simulink library "halin"  (R2024a)
settings: Solver=VariableStepAuto  StartTime=0.0  StopTime=10.0  RelTol=1e-3
undefined symbols (not defined in the file): KHAL_CAN3BMS1E2E_flg, KHAL_CAN3BMS6E2E_flg, TimeoutOccurred
libraries: FVT_lib x12, simulink x6, hcu_lib x1
(part 1 of 2)
settings Model: Creator=13168  LastModifiedBy=FVT22063
settings SolverCC: AlgebraicLoopSolver=TrustRegion
settings DataIOCC: SaveFormat=Array  SignalLoggingSaveFormat=ModelDataLogs  ReturnWorkspaceOutputs=off
settings OptimizationCC: BlockReduction=off  BooleanDataType=off
settings DebuggingCC: SaveWithParameterizedLinksMsg=none  UnderspecifiedInitializationDetection=Classic  MergeDetectMultiDrivingBlocksExec=none  SignalResolutionControl=TryResolveAllWithWarning  UnconnectedInputMsg=warning  UnconnectedOutputMsg=warning  UnconnectedLineMsg=warning
settings HardwareCC: TargetUnknown=on
settings ModelReferenceCC: EnableRefExpFcnMdlSchedulingChecks=on  PropagateSignalLabelsOutOfModel=off
settings RTWCC: GPUComputeCapability=3.5  DLArmComputeVersion=19.05
settings ConfigComp: CovMetricSettings=dw  CovSaveCumulativeToWorkspaceVar=on  CovSaveSingleToWorkspaceVar=on

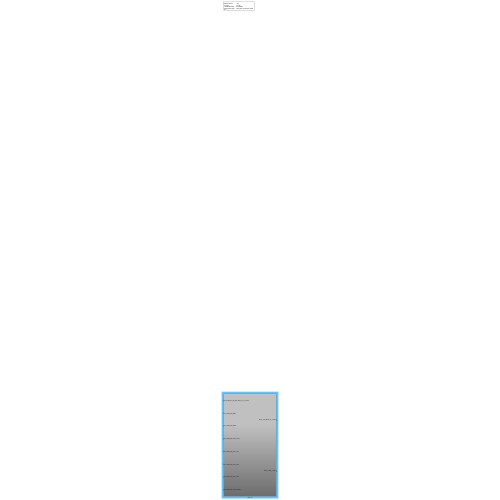
[thumbnail: Simulink's stored preview of the top-level diagram]
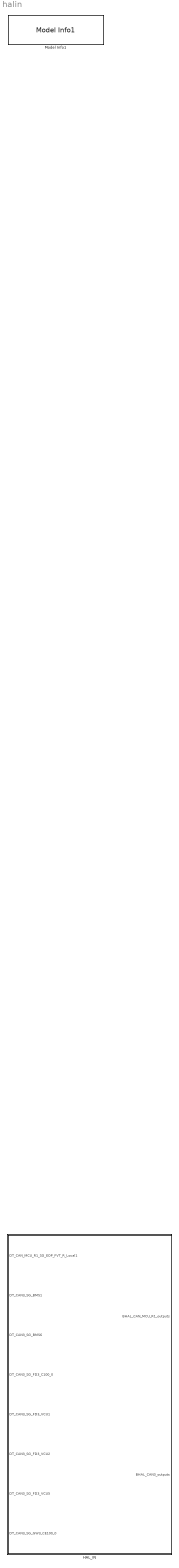
== system halin ==
  HAL_IN : Subsystem
      settings: RTWSystemCode=Nonreusable function  RTWFcnNameOpts=Use subsystem name  RTWFileNameOpts=Use subsystem name
  Model Info1 : hcu_lib/Model Info1  BlockCM=None  Frame=on  DisplayStringWithTags=|  HorizontalTextAlignment=Left  LeftAlignmentValue=0.02  SourceBlockDiagram=hcu_lib  TagMaxNumber=20
      | Model Version        : %<ModelVersion>
      | Creator                   : %<Creator>
      | Last Modified By    : %<LastModifiedBy>
      | Modification date    : %<LastModificationDate>
      settings: SourceProductName=HCU Relative Block Library

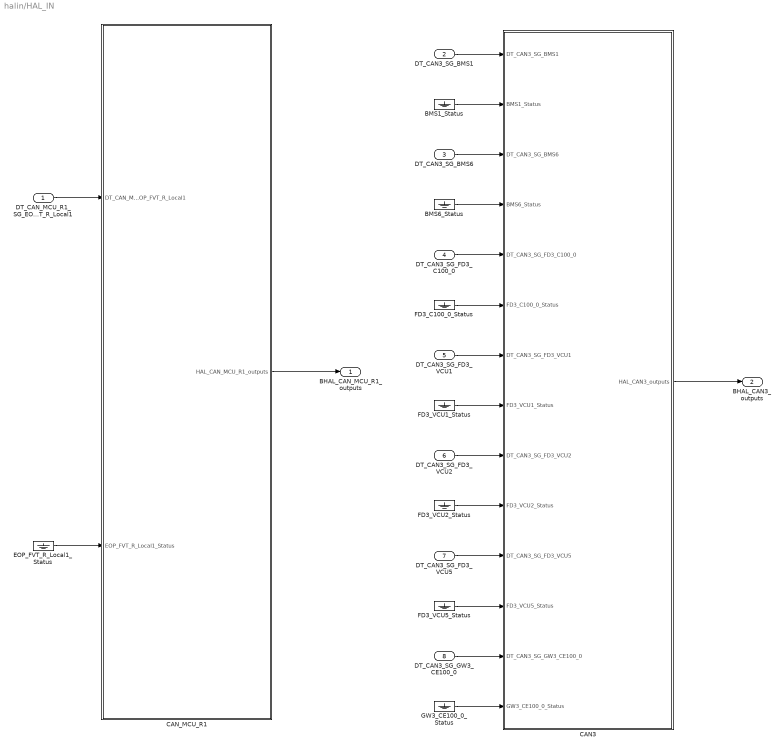
== system halin/HAL_IN ==
  DT_CAN_MCU_R1_SG_EOP_FVT_R_Local1 : Inport
  DT_CAN3_SG_BMS1 : Inport  Port=2
  DT_CAN3_SG_BMS6 : Inport  Port=3
  DT_CAN3_SG_FD3_C100_0 : Inport  Port=4
  DT_CAN3_SG_FD3_VCU1 : Inport  Port=5
  DT_CAN3_SG_FD3_VCU2 : Inport  Port=6
  DT_CAN3_SG_FD3_VCU5 : Inport  Port=7
  DT_CAN3_SG_GW3_CE100_0 : Inport  Port=8
  BMS1_Status : Ground
  BMS6_Status : Ground
  CAN3 : Subsystem
  CAN_MCU_R1 : Subsystem
  EOP_FVT_R_Local1_Status : Ground
  FD3_C100_0_Status : Ground
  FD3_VCU1_Status : Ground
  FD3_VCU2_Status : Ground
  FD3_VCU5_Status : Ground
  GW3_CE100_0_Status : Ground
  BHAL_CAN_MCU_R1_outputs : Outport  OutDataTypeStr=Bus: BHAL_CAN_MCU_R1_outputs
  BHAL_CAN3_outputs : Outport  Port=2  OutDataTypeStr=Bus: BHAL_CAN3_outputs
  wires:
  GW3_CE100_0_Status/1 -> CAN3/14(GW3_CE100_0_Status)
  DT_CAN3_SG_GW3_CE100_0/1 -> CAN3/13(DT_CAN3_SG_GW3_CE100_0)
  FD3_VCU5_Status/1 -> CAN3/12(FD3_VCU5_Status)
  DT_CAN3_SG_FD3_VCU5/1 -> CAN3/11(DT_CAN3_SG_FD3_VCU5)
  DT_CAN3_SG_FD3_VCU2/1 -> CAN3/9(DT_CAN3_SG_FD3_VCU2)
  FD3_VCU2_Status/1 -> CAN3/10(FD3_VCU2_Status)
  FD3_VCU1_Status/1 -> CAN3/8(FD3_VCU1_Status)
  FD3_C100_0_Status/1 -> CAN3/6(FD3_C100_0_Status)
  DT_CAN3_SG_FD3_VCU1/1 -> CAN3/7(DT_CAN3_SG_FD3_VCU1)
  DT_CAN3_SG_FD3_C100_0/1 -> CAN3/5(DT_CAN3_SG_FD3_C100_0)
  DT_CAN3_SG_BMS6/1 -> CAN3/3(DT_CAN3_SG_BMS6)
  BMS6_Status/1 -> CAN3/4(BMS6_Status)
  CAN3/1(HAL_CAN3_outputs) -> BHAL_CAN3_outputs/1
  BMS1_Status/1 -> CAN3/2(BMS1_Status)
  CAN_MCU_R1/1(HAL_CAN_MCU_R1_outputs) -> BHAL_CAN_MCU_R1_outputs/1
  EOP_FVT_R_Local1_Status/1 -> CAN_MCU_R1/2(EOP_FVT_R_Local1_Status)
  DT_CAN3_SG_BMS1/1 -> CAN3/1(DT_CAN3_SG_BMS1)
  DT_CAN_MCU_R1_SG_EOP_FVT_R_Local1/1 -> CAN_MCU_R1/1(DT_CAN_MCU_R1_SG_EOP_FVT_R_Local1)

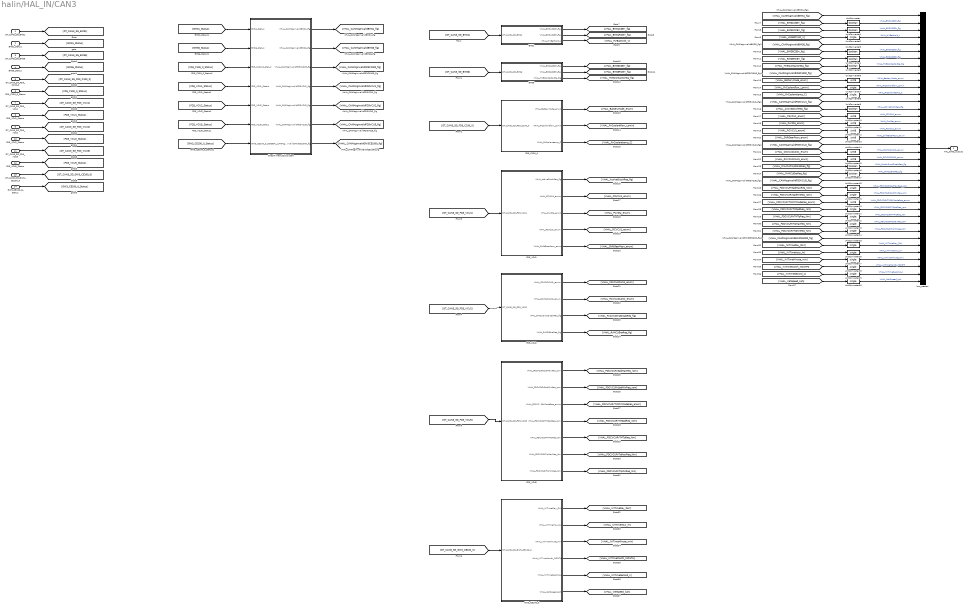
== system halin/HAL_IN/CAN3 ==
  DT_CAN3_SG_BMS1 : Inport
  BMS1_Status : Inport  Port=2
  DT_CAN3_SG_BMS6 : Inport  Port=3
  BMS6_Status : Inport  Port=4
  DT_CAN3_SG_FD3_C100_0 : Inport  Port=5
  FD3_C100_0_Status : Inport  Port=6
  DT_CAN3_SG_FD3_VCU1 : Inport  Port=7
  FD3_VCU1_Status : Inport  Port=8
  DT_CAN3_SG_FD3_VCU2 : Inport  Port=9
  FD3_VCU2_Status : Inport  Port=10
  DT_CAN3_SG_FD3_VCU5 : Inport  Port=11
  FD3_VCU5_Status : Inport  Port=12
  DT_CAN3_SG_GW3_CE100_0 : Inport  Port=13
  GW3_CE100_0_Status : Inport  Port=14
  BMS1 : Subsystem
  BMS6 : Subsystem
  CheckTimeoutSubsystem : Subsystem
  FD3_C100_0 : Subsystem
  FD3_VCU1 : Subsystem
  FD3_VCU2 : Subsystem
  FD3_VCU5 : Subsystem
  GW3_CE100_0 : Subsystem
  UnitConverter{,1,3..5,9,16..17} (8 alike) : DataTypeConversion  OutDataTypeStr=boolean  SaturateOnIntegerOverflow=off  RndMeth=Floor
  UnitConverter{6,10..15,20} (8 alike) : DataTypeConversion  OutDataTypeStr=uint8  SaturateOnIntegerOverflow=off  RndMeth=Floor
  UnitConverter{2,7..8,18..19,21..30} (15 alike) : DataTypeConversion  OutDataTypeStr=single  SaturateOnIntegerOverflow=off  RndMeth=Floor
  bus_creator : BusCreator  Inputs=38  OutDataTypeStr=Bus: BHAL_CAN3_outputs  NonVirtualBus=on
  HAL_CAN3_outputs : Outport
  wires:
  BMS1_Status/1 -> [BMS1_Status]
  DT_CAN3_SG_BMS1/1 -> [DT_CAN3_SG_BMS1]
  BMS6_Status/1 -> [BMS6_Status]
  DT_CAN3_SG_BMS6/1 -> [DT_CAN3_SG_BMS6]
  FD3_C100_0_Status/1 -> [FD3_C100_0_Status]
  DT_CAN3_SG_FD3_C100_0/1 -> [DT_CAN3_SG_FD3_C100_0]
  FD3_VCU1_Status/1 -> [FD3_VCU1_Status]
  DT_CAN3_SG_FD3_VCU1/1 -> [DT_CAN3_SG_FD3_VCU1]
  FD3_VCU2_Status/1 -> [FD3_VCU2_Status]
  DT_CAN3_SG_FD3_VCU2/1 -> [DT_CAN3_SG_FD3_VCU2]
  FD3_VCU5_Status/1 -> [FD3_VCU5_Status]
  DT_CAN3_SG_FD3_VCU5/1 -> [DT_CAN3_SG_FD3_VCU5]
  GW3_CE100_0_Status/1 -> [GW3_CE100_0_Status]
  DT_CAN3_SG_GW3_CE100_0/1 -> [DT_CAN3_SG_GW3_CE100_0]
  [BMS1_Status] -> CheckTimeoutSubsystem/1(BMS1_Status)
  [BMS6_Status] -> CheckTimeoutSubsystem/2(BMS6_Status)
  [FD3_C100_0_Status] -> CheckTimeoutSubsystem/3(FD3_C100_0_Status)
  [FD3_VCU1_Status] -> CheckTimeoutSubsystem/4(FD3_VCU1_Status)
  [FD3_VCU2_Status] -> CheckTimeoutSubsystem/5(FD3_VCU2_Status)
  [FD3_VCU5_Status] -> CheckTimeoutSubsystem/6(FD3_VCU5_Status)
  [GW3_CE100_0_Status] -> CheckTimeoutSubsystem/7(GW3_CE100_0_Status)
  CheckTimeoutSubsystem/1(VHAL_CANMsgInvalidBMS1_flg) -> [VHAL_CANMsgInvalidBMS1_flg]
  CheckTimeoutSubsystem/2(VHAL_CANMsgInvalidBMS6_flg) -> [VHAL_CANMsgInvalidBMS6_flg]
  CheckTimeoutSubsystem/3(VHAL_CANMsgInvalidFD3C1000_flg) -> [VHAL_CANMsgInvalidFD3C1000_flg]
  CheckTimeoutSubsystem/4(VHAL_CANMsgInvalidFD3VCU1_flg) -> [VHAL_CANMsgInvalidFD3VCU1_flg]
  CheckTimeoutSubsystem/5(VHAL_CANMsgInvalidFD3VCU2_flg) -> [VHAL_CANMsgInvalidFD3VCU2_flg]
  CheckTimeoutSubsystem/6(VHAL_CANMsgInvalidFD3VCU5_flg) -> [VHAL_CANMsgInvalidFD3VCU5_flg]
  CheckTimeoutSubsystem/7(VHAL_CANMsgInvalidGW3CE1000_flg) -> [VHAL_CANMsgInvalidGW3CE1000_flg]
  [DT_CAN3_SG_BMS1] -> BMS1/1(DT_CAN3_SG_BMS1)
  [DT_CAN3_SG_BMS6] -> BMS6/1(DT_CAN3_SG_BMS6)
  [DT_CAN3_SG_FD3_C100_0] -> FD3_C100_0/1(DT_CAN3_SG_FD3_C100_0)
  [DT_CAN3_SG_FD3_VCU1] -> FD3_VCU1/1(DT_CAN3_SG_FD3_VCU1)
  [DT_CAN3_SG_FD3_VCU2] -> FD3_VCU2/1(DT_CAN3_SG_FD3_VCU2)
  [DT_CAN3_SG_FD3_VCU5] -> FD3_VCU5/1(DT_CAN3_SG_FD3_VCU5)
  [DT_CAN3_SG_GW3_CE100_0] -> GW3_CE100_0/1(DT_CAN3_SG_GW3_CE100_0)
  bus_creator/1 -> HAL_CAN3_outputs/1
  [VHAL_CANMsgInvalidBMS1_flg] -> bus_creator/1
  BMS1/1(VHAL_BMS1CSErr_flg) -> [VHAL_BMS1CSErr_flg]
  UnitConverter/1 -> bus_creator/2  "VHAL_BMS1CSErr_flg"
  [VHAL_BMS1CSErr_flg] -> UnitConverter/1
  BMS1/2(VHAL_BMS1RCErr_flg) -> [VHAL_BMS1RCErr_flg]
  UnitConverter1/1 -> bus_creator/3  "VHAL_BMS1RCErr_flg"
  [VHAL_BMS1RCErr_flg] -> UnitConverter1/1
  BMS1/3(VHAL_HVBattVolt_V) -> [VHAL_HVBattVolt_V]
  UnitConverter2/1 -> bus_creator/4  "VHAL_HVBattVolt_V"
  [VHAL_HVBattVolt_V] -> UnitConverter2/1
  [VHAL_CANMsgInvalidBMS6_flg] -> bus_creator/5
  BMS6/1(VHAL_BMS6CSErr_flg) -> [VHAL_BMS6CSErr_flg]
  UnitConverter3/1 -> bus_creator/6  "VHAL_BMS6CSErr_flg"
  [VHAL_BMS6CSErr_flg] -> UnitConverter3/1
  BMS6/2(VHAL_BMS6RCErr_flg) -> [VHAL_BMS6RCErr_flg]
  UnitConverter4/1 -> bus_creator/7  "VHAL_BMS6RCErr_flg"
  [VHAL_BMS6RCErr_flg] -> UnitConverter4/1
  BMS6/3(VHAL_HVBContactorSta_flg) -> [VHAL_HVBContactorSta_flg]
  UnitConverter5/1 -> bus_creator/8  "VHAL_HVBContactorSta_flg"
  [VHAL_HVBContactorSta_flg] -> UnitConverter5/1
  [VHAL_CANMsgInvalidFD3C1000_flg] -> bus_creator/9
  FD3_C100_0/1(VHAL_BatteryMode_enum) -> [VHAL_BatteryMode_enum]
  UnitConverter6/1 -> bus_creator/10  "VHAL_BatteryMode_enum"
  [VHAL_BatteryMode_enum] -> UnitConverter6/1
  FD3_C100_0/2(VHAL_RrCoolantflow_Lpmin) -> [VHAL_RrCoolantflow_Lpmin]
  UnitConverter7/1 -> bus_creator/11  "VHAL_RrCoolantflow_Lpmin"
  [VHAL_RrCoolantflow_Lpmin] -> UnitConverter7/1
  FD3_C100_0/3(VHAL_RrCoolanttemp_C) -> [VHAL_RrCoolanttemp_C]
  UnitConverter8/1 -> bus_creator/12  "VHAL_RrCoolanttemp_C"
  [VHAL_RrCoolanttemp_C] -> UnitConverter8/1
  [VHAL_CANMsgInvalidFD3VCU1_flg] -> bus_creator/13
  FD3_VCU1/1(VHAL_ActiveDischReq_flg) -> [VHAL_ActiveDischReq_flg]
  UnitConverter9/1 -> bus_creator/14  "VHAL_ActiveDischReq_flg"
  [VHAL_ActiveDischReq_flg] -> UnitConverter9/1
  FD3_VCU1/2(VHAL_CSVCU1_enum) -> [VHAL_CSVCU1_enum]
  UnitConverter10/1 -> bus_creator/15  "VHAL_CSVCU1_enum"
  [VHAL_CSVCU1_enum] -> UnitConverter10/1
  FD3_VCU1/3(VHAL_PwrSta_enum) -> [VHAL_PwrSta_enum]
  UnitConverter11/1 -> bus_creator/16  "VHAL_PwrSta_enum"
  [VHAL_PwrSta_enum] -> UnitConverter11/1
  FD3_VCU1/4(VHAL_RCVCU1_enum) -> [VHAL_RCVCU1_enum]
  UnitConverter12/1 -> bus_creator/17  "VHAL_RCVCU1_enum"
  [VHAL_RCVCU1_enum] -> UnitConverter12/1
  FD3_VCU1/5(VHAL_ShiftGearPosn_enum) -> [VHAL_ShiftGearPosn_enum]
  UnitConverter13/1 -> bus_creator/18  "VHAL_ShiftGearPosn_enum"
  [VHAL_ShiftGearPosn_enum] -> UnitConverter13/1
  [VHAL_CANMsgInvalidFD3VCU2_flg] -> bus_creator/19
  FD3_VCU2/1(VHAL_CSVCU2CAN1_enum) -> [VHAL_CSVCU2CAN1_enum]
  UnitConverter14/1 -> bus_creator/20  "VHAL_CSVCU2CAN1_enum"
  [VHAL_CSVCU2CAN1_enum] -> UnitConverter14/1
  FD3_VCU2/2(VHAL_RCVCU2CAN1_enum) -> [VHAL_RCVCU2CAN1_enum]
  UnitConverter15/1 -> bus_creator/21  "VHAL_RCVCU2CAN1_enum"
  [VHAL_RCVCU2CAN1_enum] -> UnitConverter15/1
  FD3_VCU2/3(VHAL_RrActvDmpDisabReq_flg) -> [VHAL_RrActvDmpDisabReq_flg]
  UnitConverter16/1 -> bus_creator/22  "VHAL_RrActvDmpDisabReq_flg"
  [VHAL_RrActvDmpDisabReq_flg] -> UnitConverter16/1
  FD3_VCU2/4(VHAL_RrMCUEnaReq_flg) -> [VHAL_RrMCUEnaReq_flg]
  UnitConverter17/1 -> bus_creator/23  "VHAL_RrMCUEnaReq_flg"
  [VHAL_RrMCUEnaReq_flg] -> UnitConverter17/1
  [VHAL_CANMsgInvalidFD3VCU5_flg] -> bus_creator/24
  FD3_VCU5/1(VHAL_FDCVCURrSpdMaxReq_rpm) -> [VHAL_FDCVCURrSpdMaxReq_rpm]
  UnitConverter18/1 -> bus_creator/25  "VHAL_FDCVCURrSpdMaxReq_rpm"
  [VHAL_FDCVCURrSpdMaxReq_rpm] -> UnitConverter18/1
  FD3_VCU5/2(VHAL_FDCVCURrSpdMinReq_rpm) -> [VHAL_FDCVCURrSpdMinReq_rpm]
  UnitConverter19/1 -> bus_creator/26  "VHAL_FDCVCURrSpdMinReq_rpm"
  [VHAL_FDCVCURrSpdMinReq_rpm] -> UnitConverter19/1
  FD3_VCU5/3(VHAL_FDCVCURrTMCtrlModeReq_enum) -> [VHAL_FDCVCURrTMCtrlModeReq_enum]
  UnitConverter20/1 -> bus_creator/27  "VHAL_FDCVCURrTMCtrlModeReq_enum"
  [VHAL_FDCVCURrTMCtrlModeReq_enum] -> UnitConverter20/1
  FD3_VCU5/4(VHAL_FDCVCURrTMSpdReq_rpm) -> [VHAL_FDCVCURrTMSpdReq_rpm]
  UnitConverter21/1 -> bus_creator/28  "VHAL_FDCVCURrTMSpdReq_rpm"
  [VHAL_FDCVCURrTMSpdReq_rpm] -> UnitConverter21/1
  FD3_VCU5/5(VHAL_FDCVCURrTMTqReq_Nm) -> [VHAL_FDCVCURrTMTqReq_Nm]
  UnitConverter22/1 -> bus_creator/29  "VHAL_FDCVCURrTMTqReq_Nm"
  [VHAL_FDCVCURrTMTqReq_Nm] -> UnitConverter22/1
  FD3_VCU5/6(VHAL_FDCVCURrTqMaxReq_Nm) -> [VHAL_FDCVCURrTqMaxReq_Nm]
  UnitConverter23/1 -> bus_creator/30  "VHAL_FDCVCURrTqMaxReq_Nm"
  [VHAL_FDCVCURrTqMaxReq_Nm] -> UnitConverter23/1
  FD3_VCU5/7(VHAL_FDCVCURrTqMinReq_Nm) -> [VHAL_FDCVCURrTqMinReq_Nm]
  UnitConverter24/1 -> bus_creator/31  "VHAL_FDCVCURrTqMinReq_Nm"
  [VHAL_FDCVCURrTqMinReq_Nm] -> UnitConverter24/1
  [VHAL_CANMsgInvalidGW3CE1000_flg] -> bus_creator/32
  GW3_CE100_0/1(VHAL_IVITimeDay_DAY) -> [VHAL_IVITimeDay_DAY]
  UnitConverter25/1 -> bus_creator/33  "VHAL_IVITimeDay_DAY"
  [VHAL_IVITimeDay_DAY] -> UnitConverter25/1
  GW3_CE100_0/2(VHAL_IVITimeHour_hr) -> [VHAL_IVITimeHour_hr]
  UnitConverter26/1 -> bus_creator/34  "VHAL_IVITimeHour_hr"
  [VHAL_IVITimeHour_hr] -> UnitConverter26/1
  GW3_CE100_0/3(VHAL_IVITimeMinute_min) -> [VHAL_IVITimeMinute_min]
  UnitConverter27/1 -> bus_creator/35  "VHAL_IVITimeMinute_min"
  [VHAL_IVITimeMinute_min] -> UnitConverter27/1
  GW3_CE100_0/4(VHAL_IVITimeMonth_MONTH) -> [VHAL_IVITimeMonth_MONTH]
  UnitConverter28/1 -> bus_creator/36  "VHAL_IVITimeMonth_MONTH"
  [VHAL_IVITimeMonth_MONTH] -> UnitConverter28/1
  GW3_CE100_0/5(VHAL_IVITimeSecond_s) -> [VHAL_IVITimeSecond_s]
  UnitConverter29/1 -> bus_creator/37  "VHAL_IVITimeSecond_s"
  [VHAL_IVITimeSecond_s] -> UnitConverter29/1
  GW3_CE100_0/6(VHAL_VehSpeed_kph) -> [VHAL_VehSpeed_kph]
  UnitConverter30/1 -> bus_creator/38  "VHAL_VehSpeed_kph"
  [VHAL_VehSpeed_kph] -> UnitConverter30/1

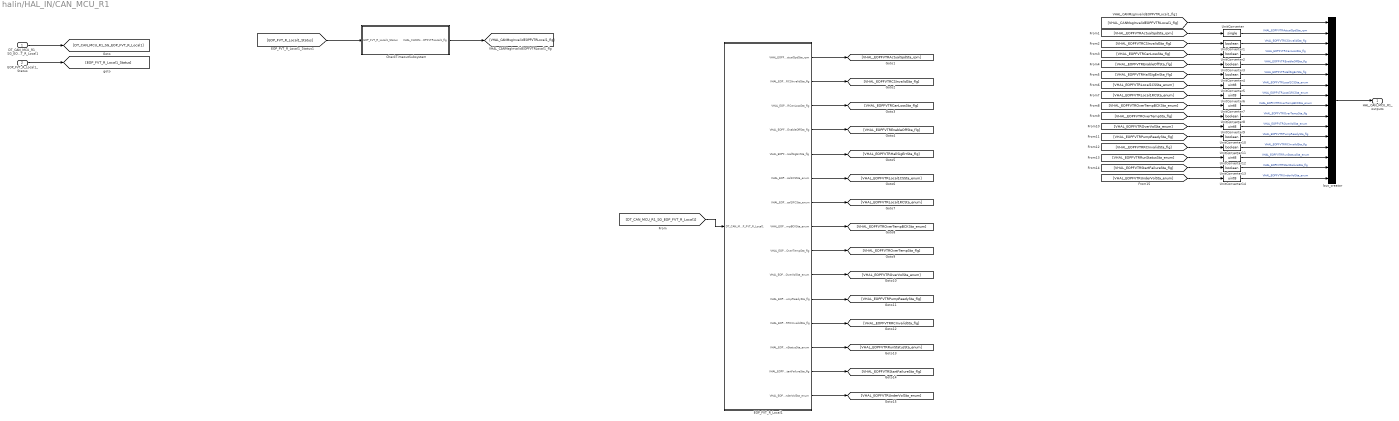
== system halin/HAL_IN/CAN_MCU_R1 ==
  DT_CAN_MCU_R1_SG_EOP_FVT_R_Local1 : Inport
  EOP_FVT_R_Local1_Status : Inport  Port=2
  CheckTimeoutSubsystem : Subsystem
  EOP_FVT_R_Local1 : Subsystem
  UnitConverter : DataTypeConversion  OutDataTypeStr=single  SaturateOnIntegerOverflow=off  RndMeth=Floor
  UnitConverter{1..4,8,10..11,13} (8 alike) : DataTypeConversion  OutDataTypeStr=boolean  SaturateOnIntegerOverflow=off  RndMeth=Floor
  UnitConverter{5..7,9,12,14} (6 alike) : DataTypeConversion  OutDataTypeStr=uint8  SaturateOnIntegerOverflow=off  RndMeth=Floor
  bus_creator : BusCreator  Inputs=16  OutDataTypeStr=Bus: BHAL_CAN_MCU_R1_outputs  NonVirtualBus=on
  HAL_CAN_MCU_R1_outputs : Outport
  wires:
  EOP_FVT_R_Local1_Status/1 -> [EOP_FVT_R_Local1_Status]
  DT_CAN_MCU_R1_SG_EOP_FVT_R_Local1/1 -> [DT_CAN_MCU_R1_SG_EOP_FVT_R_Local1]
  [EOP_FVT_R_Local1_Status] -> CheckTimeoutSubsystem/1(EOP_FVT_R_Local1_Status)
  CheckTimeoutSubsystem/1(VHAL_CANMsgInvalidEOPFVTRLocal1_flg) -> [VHAL_CANMsgInvalidEOPFVTRLocal1_flg]
  [DT_CAN_MCU_R1_SG_EOP_FVT_R_Local1] -> EOP_FVT_R_Local1/1(DT_CAN_MCU_R1_SG_EOP_FVT_R_Local1)
  bus_creator/1 -> HAL_CAN_MCU_R1_outputs/1
  [VHAL_CANMsgInvalidEOPFVTRLocal1_flg] -> bus_creator/1
  EOP_FVT_R_Local1/1(VHAL_EOPFVTRActualSpdSta_rpm) -> [VHAL_EOPFVTRActualSpdSta_rpm]
  UnitConverter/1 -> bus_creator/2  "VHAL_EOPFVTRActualSpdSta_rpm"
  [VHAL_EOPFVTRActualSpdSta_rpm] -> UnitConverter/1
  EOP_FVT_R_Local1/2(VHAL_EOPFVTRCSInvalidSta_flg) -> [VHAL_EOPFVTRCSInvalidSta_flg]
  UnitConverter1/1 -> bus_creator/3  "VHAL_EOPFVTRCSInvalidSta_flg"
  [VHAL_EOPFVTRCSInvalidSta_flg] -> UnitConverter1/1
  EOP_FVT_R_Local1/3(VHAL_EOPFVTRCanLossSta_flg) -> [VHAL_EOPFVTRCanLossSta_flg]
  UnitConverter2/1 -> bus_creator/4  "VHAL_EOPFVTRCanLossSta_flg"
  [VHAL_EOPFVTRCanLossSta_flg] -> UnitConverter2/1
  EOP_FVT_R_Local1/4(VHAL_EOPFVTREnableOffSta_flg) -> [VHAL_EOPFVTREnableOffSta_flg]
  UnitConverter3/1 -> bus_creator/5  "VHAL_EOPFVTREnableOffSta_flg"
  [VHAL_EOPFVTREnableOffSta_flg] -> UnitConverter3/1
  EOP_FVT_R_Local1/5(VHAL_EOPFVTRHallSigErrSta_flg) -> [VHAL_EOPFVTRHallSigErrSta_flg]
  UnitConverter4/1 -> bus_creator/6  "VHAL_EOPFVTRHallSigErrSta_flg"
  [VHAL_EOPFVTRHallSigErrSta_flg] -> UnitConverter4/1
  EOP_FVT_R_Local1/6(VHAL_EOPFVTRLocal1CSSta_enum) -> [VHAL_EOPFVTRLocal1CSSta_enum]
  UnitConverter5/1 -> bus_creator/7  "VHAL_EOPFVTRLocal1CSSta_enum"
  [VHAL_EOPFVTRLocal1CSSta_enum] -> UnitConverter5/1
  EOP_FVT_R_Local1/7(VHAL_EOPFVTRLocal1RCSta_enum) -> [VHAL_EOPFVTRLocal1RCSta_enum]
  UnitConverter6/1 -> bus_creator/8  "VHAL_EOPFVTRLocal1RCSta_enum"
  [VHAL_EOPFVTRLocal1RCSta_enum] -> UnitConverter6/1
  EOP_FVT_R_Local1/8(VHAL_EOPFVTROverTempBCKSta_enum) -> [VHAL_EOPFVTROverTempBCKSta_enum]
  UnitConverter7/1 -> bus_creator/9  "VHAL_EOPFVTROverTempBCKSta_enum"
  [VHAL_EOPFVTROverTempBCKSta_enum] -> UnitConverter7/1
  EOP_FVT_R_Local1/9(VHAL_EOPFVTROverTempSta_flg) -> [VHAL_EOPFVTROverTempSta_flg]
  UnitConverter8/1 -> bus_creator/10  "VHAL_EOPFVTROverTempSta_flg"
  [VHAL_EOPFVTROverTempSta_flg] -> UnitConverter8/1
  EOP_FVT_R_Local1/10(VHAL_EOPFVTROverVolSta_enum) -> [VHAL_EOPFVTROverVolSta_enum]
  UnitConverter9/1 -> bus_creator/11  "VHAL_EOPFVTROverVolSta_enum"
  [VHAL_EOPFVTROverVolSta_enum] -> UnitConverter9/1
  EOP_FVT_R_Local1/11(VHAL_EOPFVTRPumpReadySta_flg) -> [VHAL_EOPFVTRPumpReadySta_flg]
  UnitConverter10/1 -> bus_creator/12  "VHAL_EOPFVTRPumpReadySta_flg"
  [VHAL_EOPFVTRPumpReadySta_flg] -> UnitConverter10/1
  EOP_FVT_R_Local1/12(VHAL_EOPFVTRRCInvalidSta_flg) -> [VHAL_EOPFVTRRCInvalidSta_flg]
  UnitConverter11/1 -> bus_creator/13  "VHAL_EOPFVTRRCInvalidSta_flg"
  [VHAL_EOPFVTRRCInvalidSta_flg] -> UnitConverter11/1
  EOP_FVT_R_Local1/13(VHAL_EOPFVTRRunStatusSta_enum) -> [VHAL_EOPFVTRRunStatusSta_enum]
  UnitConverter12/1 -> bus_creator/14  "VHAL_EOPFVTRRunStatusSta_enum"
  [VHAL_EOPFVTRRunStatusSta_enum] -> UnitConverter12/1
  EOP_FVT_R_Local1/14(VHAL_EOPFVTRStartFailureSta_flg) -> [VHAL_EOPFVTRStartFailureSta_flg]
  UnitConverter13/1 -> bus_creator/15  "VHAL_EOPFVTRStartFailureSta_flg"
  [VHAL_EOPFVTRStartFailureSta_flg] -> UnitConverter13/1
  EOP_FVT_R_Local1/15(VHAL_EOPFVTRUnderVolSta_enum) -> [VHAL_EOPFVTRUnderVolSta_enum]
  UnitConverter14/1 -> bus_creator/16  "VHAL_EOPFVTRUnderVolSta_enum"
  [VHAL_EOPFVTRUnderVolSta_enum] -> UnitConverter14/1

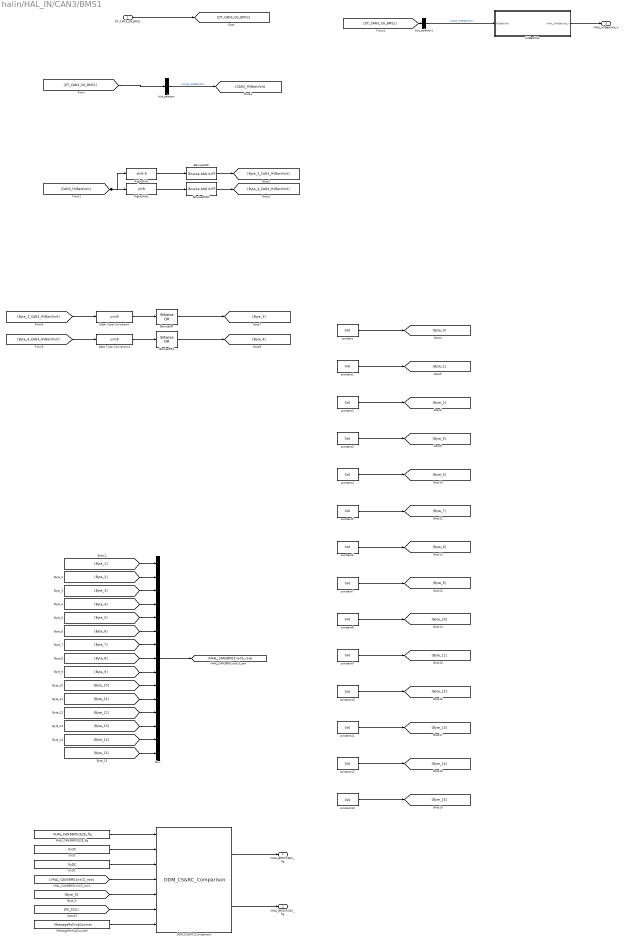
== system halin/HAL_IN/CAN3/BMS1 ==
  DT_CAN3_SG_BMS1 : Inport
  0x3C : Constant  Value=0x3C
  0xDC : Constant  Value=0xDC
  BitwiseAND : simulink/Logic and Bit Operations/Bitwise Operator  logicop=AND  UseBitMask=on  BitMask=0xFF  BitMaskRealWorld=Stored Integer
  BitwiseAND1 : simulink/Logic and Bit Operations/Bitwise Operator  logicop=AND  UseBitMask=on  BitMask=0xFF  BitMaskRealWorld=Stored Integer
  BitwiseOR : simulink/Logic and Bit Operations/Bitwise Operator  logicop=OR  UseBitMask=off  BitMask=bin2dec('11011001')  BitMaskRealWorld=Stored Integer
  BitwiseOR1 : simulink/Logic and Bit Operations/Bitwise Operator  logicop=OR  UseBitMask=off  BitMask=bin2dec('11011001')  BitMaskRealWorld=Stored Integer
  DDM_CS&RC_Comparison : FVT_lib/hal/DDM_CS&RC_Comparison  MsgCycleTime=10
  Data Type Conversion : DataTypeConversion  OutDataTypeStr=uint8  SaturateOnIntegerOverflow=off  RndMeth=Floor
  Data Type Conversion1 : DataTypeConversion  OutDataTypeStr=uint8  SaturateOnIntegerOverflow=off  RndMeth=Floor
  HVBattVolt : Subsystem
  KHAL_CAN3BMS1E2E_flg : Constant  Value=KHAL_CAN3BMS1E2E_flg
  MessageRollingCounter : FVT_lib/hal/MessageRollingCounter  CounterMAX=14  task_time_ms=5  msg_time_ms=10
  Mux : Mux  Inputs=15
  RightShift : ArithShift  BitShiftNumber=8
  RightShift1 : ArithShift
  bus_selector : BusSelector  OutputSignals=CAN3_HVBattVolt
  bus_selector1 : BusSelector  OutputSignals=CAN3_HVBattVolt
  constant{,1..13} (14 alike) : Constant  Value=0x0  OutDataTypeStr=uint8
  VHAL_BMS1CSErr_flg : Outport
  VHAL_BMS1RCErr_flg : Outport  Port=2
  VHAL_HVBattVolt_V : Outport  Port=3
  wires:
  DT_CAN3_SG_BMS1/1 -> [DT_CAN3_SG_BMS1]
  [DT_CAN3_SG_BMS1] -> bus_selector/1
  bus_selector/1 -> [CAN3_HVBattVolt]  "<CAN3_HVBattVolt>"
  [CAN3_HVBattVolt] -> RightShift/1, RightShift1/1
  RightShift/1 -> BitwiseAND/1
  BitwiseAND/1 -> [Byte_3_CAN3_HVBattVolt]
  RightShift1/1 -> BitwiseAND1/1
  BitwiseAND1/1 -> [Byte_4_CAN3_HVBattVolt]
  constant/1 -> [Byte_0]
  constant1/1 -> [Byte_1]
  constant2/1 -> [Byte_2]
  Data Type Conversion/1 -> BitwiseOR/1
  [Byte_3_CAN3_HVBattVolt] -> Data Type Conversion/1
  BitwiseOR/1 -> [Byte_3]
  Data Type Conversion1/1 -> BitwiseOR1/1
  [Byte_4_CAN3_HVBattVolt] -> Data Type Conversion1/1
  BitwiseOR1/1 -> [Byte_4]
  constant3/1 -> [Byte_5]
  constant4/1 -> [Byte_6]
  constant5/1 -> [Byte_7]
  constant6/1 -> [Byte_8]
  constant7/1 -> [Byte_9]
  constant8/1 -> [Byte_10]
  constant9/1 -> [Byte_11]
  constant10/1 -> [Byte_12]
  constant11/1 -> [Byte_13]
  constant12/1 -> [Byte_14]
  constant13/1 -> [Byte_15]
  [Byte_1] -> Mux/1
  [Byte_2] -> Mux/2
  [Byte_3] -> Mux/3
  [Byte_4] -> Mux/4
  [Byte_5] -> Mux/5
  [Byte_6] -> Mux/6
  [Byte_7] -> Mux/7
  [Byte_8] -> Mux/8
  [Byte_9] -> Mux/9
  [Byte_10] -> Mux/10
  [Byte_11] -> Mux/11
  [Byte_12] -> Mux/12
  [Byte_13] -> Mux/13
  [Byte_14] -> Mux/14
  [Byte_15] -> Mux/15
  Mux/1 -> [VHAL_CAN3BMS1noCS_raw]
  KHAL_CAN3BMS1E2E_flg/1 -> DDM_CS&RC_Comparison/1
  0x3C/1 -> DDM_CS&RC_Comparison/2
  0xDC/1 -> DDM_CS&RC_Comparison/3
  [VHAL_CAN3BMS1noCS_raw] -> DDM_CS&RC_Comparison/4
  [Byte_0] -> DDM_CS&RC_Comparison/5
  [RC_ECU] -> DDM_CS&RC_Comparison/6
  MessageRollingCounter/1 -> DDM_CS&RC_Comparison/7
  DDM_CS&RC_Comparison/1 -> VHAL_BMS1CSErr_flg/1
  DDM_CS&RC_Comparison/2 -> VHAL_BMS1RCErr_flg/1
  [DT_CAN3_SG_BMS1] -> bus_selector1/1
  bus_selector1/1 -> HVBattVolt/1(HVBattVolt)  "<CAN3_HVBattVolt>"
  HVBattVolt/1(VHAL_HVBattVolt_V) -> VHAL_HVBattVolt_V/1

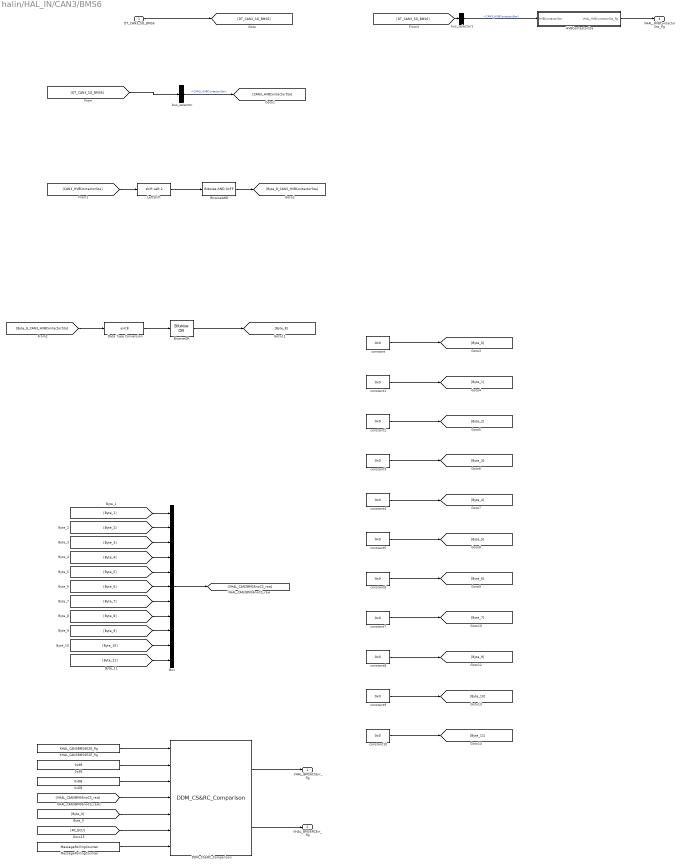
== system halin/HAL_IN/CAN3/BMS6 ==
  DT_CAN3_SG_BMS6 : Inport
  0x3B : Constant  Value=0x3B
  0xDB : Constant  Value=0xDB
  BitwiseAND : simulink/Logic and Bit Operations/Bitwise Operator  logicop=AND  UseBitMask=on  BitMask=0xFF  BitMaskRealWorld=Stored Integer
  BitwiseOR : simulink/Logic and Bit Operations/Bitwise Operator  logicop=OR  UseBitMask=off  BitMask=bin2dec('11011001')  BitMaskRealWorld=Stored Integer
  DDM_CS&RC_Comparison : FVT_lib/hal/DDM_CS&RC_Comparison  MsgCycleTime=100
  Data Type Conversion : DataTypeConversion  OutDataTypeStr=uint8  SaturateOnIntegerOverflow=off  RndMeth=Floor
  HVBContactorSta : Subsystem
  KHAL_CAN3BMS6E2E_flg : Constant  Value=KHAL_CAN3BMS6E2E_flg
  LeftShift : ArithShift  BitShiftNumber=2  BitShiftDirection=Left
  MessageRollingCounter : FVT_lib/hal/MessageRollingCounter  CounterMAX=14  task_time_ms=5  msg_time_ms=100
  Mux : Mux  Inputs=11
  bus_selector : BusSelector  OutputSignals=CAN3_HVBContactorSta
  bus_selector1 : BusSelector  OutputSignals=CAN3_HVBContactorSta
  constant{,1..10} (11 alike) : Constant  Value=0x0  OutDataTypeStr=uint8
  VHAL_BMS6CSErr_flg : Outport
  VHAL_BMS6RCErr_flg : Outport  Port=2
  VHAL_HVBContactorSta_flg : Outport  Port=3
  wires:
  DT_CAN3_SG_BMS6/1 -> [DT_CAN3_SG_BMS6]
  [DT_CAN3_SG_BMS6] -> bus_selector/1
  bus_selector/1 -> [CAN3_HVBContactorSta]  "<CAN3_HVBContactorSta>"
  [CAN3_HVBContactorSta] -> LeftShift/1
  LeftShift/1 -> BitwiseAND/1
  BitwiseAND/1 -> [Byte_8_CAN3_HVBContactorSta]
  constant/1 -> [Byte_0]
  constant1/1 -> [Byte_1]
  constant2/1 -> [Byte_2]
  constant3/1 -> [Byte_3]
  constant4/1 -> [Byte_4]
  constant5/1 -> [Byte_5]
  constant6/1 -> [Byte_6]
  constant7/1 -> [Byte_7]
  Data Type Conversion/1 -> BitwiseOR/1
  [Byte_8_CAN3_HVBContactorSta] -> Data Type Conversion/1
  BitwiseOR/1 -> [Byte_8]
  constant8/1 -> [Byte_9]
  constant9/1 -> [Byte_10]
  constant10/1 -> [Byte_11]
  [Byte_1] -> Mux/1
  [Byte_2] -> Mux/2
  [Byte_3] -> Mux/3
  [Byte_4] -> Mux/4
  [Byte_5] -> Mux/5
  [Byte_6] -> Mux/6
  [Byte_7] -> Mux/7
  [Byte_8] -> Mux/8
  [Byte_9] -> Mux/9
  [Byte_10] -> Mux/10
  [Byte_11] -> Mux/11
  Mux/1 -> [VHAL_CAN3BMS6noCS_raw]
  KHAL_CAN3BMS6E2E_flg/1 -> DDM_CS&RC_Comparison/1
  0x3B/1 -> DDM_CS&RC_Comparison/2
  0xDB/1 -> DDM_CS&RC_Comparison/3
  [VHAL_CAN3BMS6noCS_raw] -> DDM_CS&RC_Comparison/4
  [Byte_0] -> DDM_CS&RC_Comparison/5
  [RC_ECU] -> DDM_CS&RC_Comparison/6
  MessageRollingCounter/1 -> DDM_CS&RC_Comparison/7
  DDM_CS&RC_Comparison/1 -> VHAL_BMS6CSErr_flg/1
  DDM_CS&RC_Comparison/2 -> VHAL_BMS6RCErr_flg/1
  [DT_CAN3_SG_BMS6] -> bus_selector1/1
  bus_selector1/1 -> HVBContactorSta/1(HVBContactorSta)  "<CAN3_HVBContactorSta>"
  HVBContactorSta/1(VHAL_HVBContactorSta_flg) -> VHAL_HVBContactorSta_flg/1

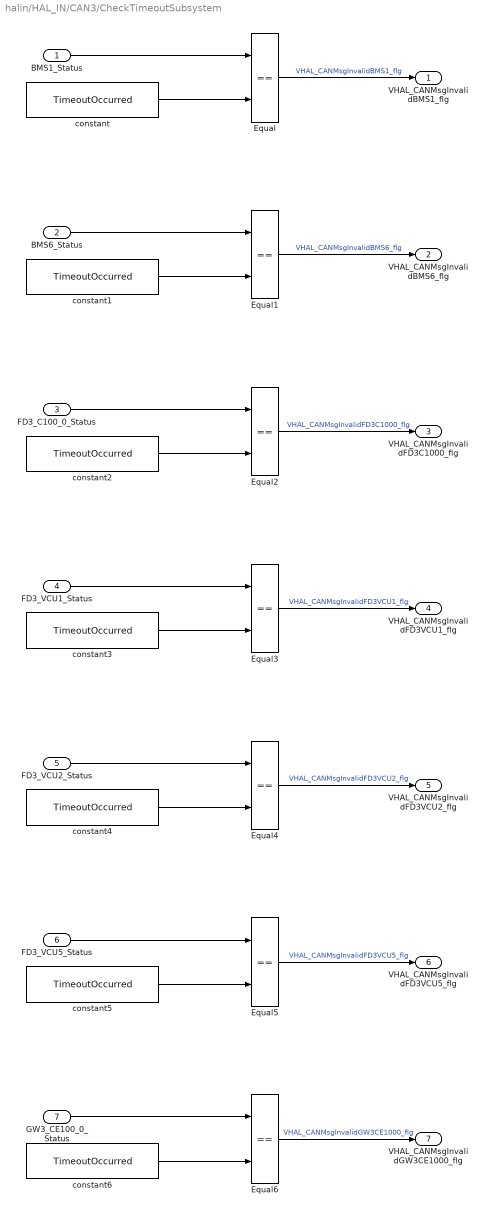
== system halin/HAL_IN/CAN3/CheckTimeoutSubsystem ==
  BMS1_Status : Inport
  BMS6_Status : Inport  Port=2
  FD3_C100_0_Status : Inport  Port=3
  FD3_VCU1_Status : Inport  Port=4
  FD3_VCU2_Status : Inport  Port=5
  FD3_VCU5_Status : Inport  Port=6
  GW3_CE100_0_Status : Inport  Port=7
  Equal{,1..6} (7 alike) : RelationalOperator  Operator===  OutDataTypeStr=boolean  RndMeth=Simplest  InputSameDT=off
  constant{,1..6} (7 alike) : Constant  Value=TimeoutOccurred
  VHAL_CANMsgInvalidBMS1_flg : Outport
  VHAL_CANMsgInvalidBMS6_flg : Outport  Port=2
  VHAL_CANMsgInvalidFD3C1000_flg : Outport  Port=3
  VHAL_CANMsgInvalidFD3VCU1_flg : Outport  Port=4
  VHAL_CANMsgInvalidFD3VCU2_flg : Outport  Port=5
  VHAL_CANMsgInvalidFD3VCU5_flg : Outport  Port=6
  VHAL_CANMsgInvalidGW3CE1000_flg : Outport  Port=7
  wires:
  BMS1_Status/1 -> Equal/1
  constant/1 -> Equal/2
  Equal/1 -> VHAL_CANMsgInvalidBMS1_flg/1  "VHAL_CANMsgInvalidBMS1_flg"
  BMS6_Status/1 -> Equal1/1
  constant1/1 -> Equal1/2
  Equal1/1 -> VHAL_CANMsgInvalidBMS6_flg/1  "VHAL_CANMsgInvalidBMS6_flg"
  FD3_C100_0_Status/1 -> Equal2/1
  constant2/1 -> Equal2/2
  Equal2/1 -> VHAL_CANMsgInvalidFD3C1000_flg/1  "VHAL_CANMsgInvalidFD3C1000_flg"
  FD3_VCU1_Status/1 -> Equal3/1
  constant3/1 -> Equal3/2
  Equal3/1 -> VHAL_CANMsgInvalidFD3VCU1_flg/1  "VHAL_CANMsgInvalidFD3VCU1_flg"
  FD3_VCU2_Status/1 -> Equal4/1
  constant4/1 -> Equal4/2
  Equal4/1 -> VHAL_CANMsgInvalidFD3VCU2_flg/1  "VHAL_CANMsgInvalidFD3VCU2_flg"
  FD3_VCU5_Status/1 -> Equal5/1
  constant5/1 -> Equal5/2
  Equal5/1 -> VHAL_CANMsgInvalidFD3VCU5_flg/1  "VHAL_CANMsgInvalidFD3VCU5_flg"
  GW3_CE100_0_Status/1 -> Equal6/1
  constant6/1 -> Equal6/2
  Equal6/1 -> VHAL_CANMsgInvalidGW3CE1000_flg/1  "VHAL_CANMsgInvalidGW3CE1000_flg"

== system halin/HAL_IN/CAN3/FD3_C100_0 ==
  DT_CAN3_SG_FD3_C100_0 : Inport
  BatteryMode : Subsystem
  RrCoolantflow : Subsystem
  RrCoolanttemp : Subsystem
  bus_selector : BusSelector  OutputSignals=CAN3_BatteryMode
  bus_selector1 : BusSelector  OutputSignals=CAN3_Rr_Coolantflow
  bus_selector2 : BusSelector  OutputSignals=CAN3_Rr_Coolanttemp
  VHAL_BatteryMode_enum : Outport
  VHAL_RrCoolantflow_Lpmin : Outport  Port=2
  VHAL_RrCoolanttemp_C : Outport  Port=3
  wires:
  DT_CAN3_SG_FD3_C100_0/1 -> [DT_CAN3_SG_FD3_C100_0]
  [DT_CAN3_SG_FD3_C100_0] -> bus_selector/1
  bus_selector/1 -> BatteryMode/1(BatteryMode)  "<CAN3_BatteryMode>"
  BatteryMode/1(VHAL_BatteryMode_enum) -> VHAL_BatteryMode_enum/1
  [DT_CAN3_SG_FD3_C100_0] -> bus_selector1/1
  bus_selector1/1 -> RrCoolantflow/1(Rr_Coolantflow)  "<CAN3_Rr_Coolantflow>"
  RrCoolantflow/1(VHAL_RrCoolantflow_Lpmin) -> VHAL_RrCoolantflow_Lpmin/1
  [DT_CAN3_SG_FD3_C100_0] -> bus_selector2/1
  bus_selector2/1 -> RrCoolanttemp/1(Rr_Coolanttemp)  "<CAN3_Rr_Coolanttemp>"
  RrCoolanttemp/1(VHAL_RrCoolanttemp_C) -> VHAL_RrCoolanttemp_C/1

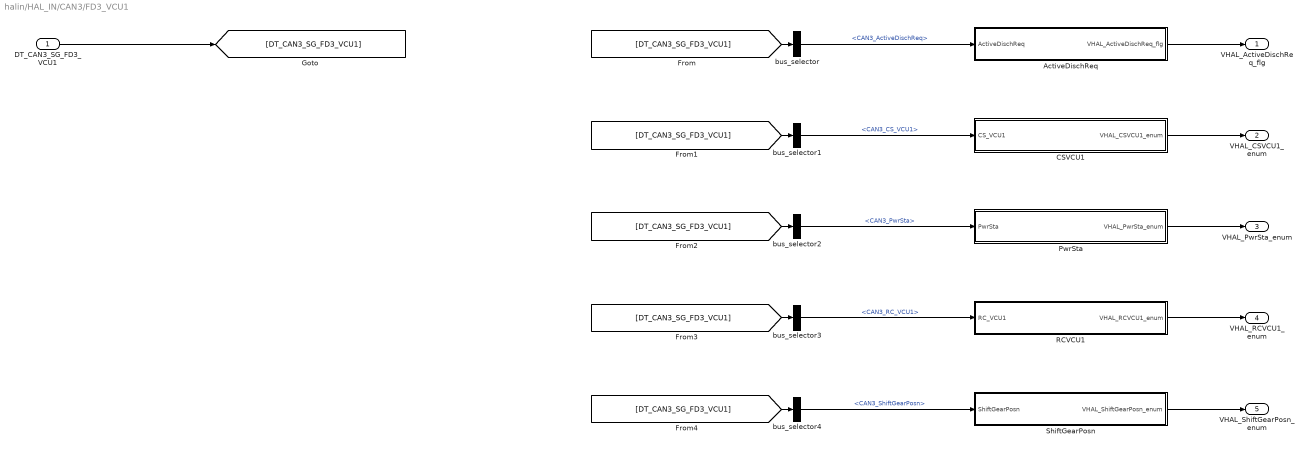
== system halin/HAL_IN/CAN3/FD3_VCU1 ==
  DT_CAN3_SG_FD3_VCU1 : Inport
  ActiveDischReq : Subsystem
  CSVCU1 : Subsystem
  PwrSta : Subsystem
  RCVCU1 : Subsystem
  ShiftGearPosn : Subsystem
  bus_selector : BusSelector  OutputSignals=CAN3_ActiveDischReq
  bus_selector1 : BusSelector  OutputSignals=CAN3_CS_VCU1
  bus_selector2 : BusSelector  OutputSignals=CAN3_PwrSta
  bus_selector3 : BusSelector  OutputSignals=CAN3_RC_VCU1
  bus_selector4 : BusSelector  OutputSignals=CAN3_ShiftGearPosn
  VHAL_ActiveDischReq_flg : Outport
  VHAL_CSVCU1_enum : Outport  Port=2
  VHAL_PwrSta_enum : Outport  Port=3
  VHAL_RCVCU1_enum : Outport  Port=4
  VHAL_ShiftGearPosn_enum : Outport  Port=5
  wires:
  DT_CAN3_SG_FD3_VCU1/1 -> [DT_CAN3_SG_FD3_VCU1]
  [DT_CAN3_SG_FD3_VCU1] -> bus_selector/1
  bus_selector/1 -> ActiveDischReq/1(ActiveDischReq)  "<CAN3_ActiveDischReq>"
  ActiveDischReq/1(VHAL_ActiveDischReq_flg) -> VHAL_ActiveDischReq_flg/1
  [DT_CAN3_SG_FD3_VCU1] -> bus_selector1/1
  bus_selector1/1 -> CSVCU1/1(CS_VCU1)  "<CAN3_CS_VCU1>"
  CSVCU1/1(VHAL_CSVCU1_enum) -> VHAL_CSVCU1_enum/1
  [DT_CAN3_SG_FD3_VCU1] -> bus_selector2/1
  bus_selector2/1 -> PwrSta/1(PwrSta)  "<CAN3_PwrSta>"
  PwrSta/1(VHAL_PwrSta_enum) -> VHAL_PwrSta_enum/1
  [DT_CAN3_SG_FD3_VCU1] -> bus_selector3/1
  bus_selector3/1 -> RCVCU1/1(RC_VCU1)  "<CAN3_RC_VCU1>"
  RCVCU1/1(VHAL_RCVCU1_enum) -> VHAL_RCVCU1_enum/1
  [DT_CAN3_SG_FD3_VCU1] -> bus_selector4/1
  bus_selector4/1 -> ShiftGearPosn/1(ShiftGearPosn)  "<CAN3_ShiftGearPosn>"
  ShiftGearPosn/1(VHAL_ShiftGearPosn_enum) -> VHAL_ShiftGearPosn_enum/1

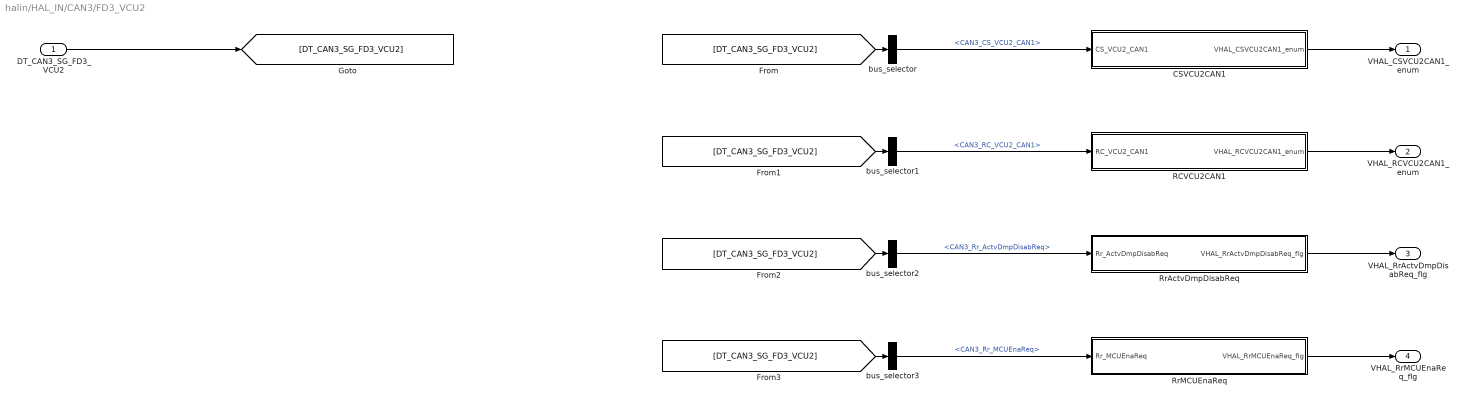
== system halin/HAL_IN/CAN3/FD3_VCU2 ==
  DT_CAN3_SG_FD3_VCU2 : Inport
  CSVCU2CAN1 : Subsystem
  RCVCU2CAN1 : Subsystem
  RrActvDmpDisabReq : Subsystem
  RrMCUEnaReq : Subsystem
  bus_selector : BusSelector  OutputSignals=CAN3_CS_VCU2_CAN1
  bus_selector1 : BusSelector  OutputSignals=CAN3_RC_VCU2_CAN1
  bus_selector2 : BusSelector  OutputSignals=CAN3_Rr_ActvDmpDisabReq
  bus_selector3 : BusSelector  OutputSignals=CAN3_Rr_MCUEnaReq
  VHAL_CSVCU2CAN1_enum : Outport
  VHAL_RCVCU2CAN1_enum : Outport  Port=2
  VHAL_RrActvDmpDisabReq_flg : Outport  Port=3
  VHAL_RrMCUEnaReq_flg : Outport  Port=4
  wires:
  DT_CAN3_SG_FD3_VCU2/1 -> [DT_CAN3_SG_FD3_VCU2]
  [DT_CAN3_SG_FD3_VCU2] -> bus_selector/1
  bus_selector/1 -> CSVCU2CAN1/1(CS_VCU2_CAN1)  "<CAN3_CS_VCU2_CAN1>"
  CSVCU2CAN1/1(VHAL_CSVCU2CAN1_enum) -> VHAL_CSVCU2CAN1_enum/1
  [DT_CAN3_SG_FD3_VCU2] -> bus_selector1/1
  bus_selector1/1 -> RCVCU2CAN1/1(RC_VCU2_CAN1)  "<CAN3_RC_VCU2_CAN1>"
  RCVCU2CAN1/1(VHAL_RCVCU2CAN1_enum) -> VHAL_RCVCU2CAN1_enum/1
  [DT_CAN3_SG_FD3_VCU2] -> bus_selector2/1
  bus_selector2/1 -> RrActvDmpDisabReq/1(Rr_ActvDmpDisabReq)  "<CAN3_Rr_ActvDmpDisabReq>"
  RrActvDmpDisabReq/1(VHAL_RrActvDmpDisabReq_flg) -> VHAL_RrActvDmpDisabReq_flg/1
  [DT_CAN3_SG_FD3_VCU2] -> bus_selector3/1
  bus_selector3/1 -> RrMCUEnaReq/1(Rr_MCUEnaReq)  "<CAN3_Rr_MCUEnaReq>"
  RrMCUEnaReq/1(VHAL_RrMCUEnaReq_flg) -> VHAL_RrMCUEnaReq_flg/1

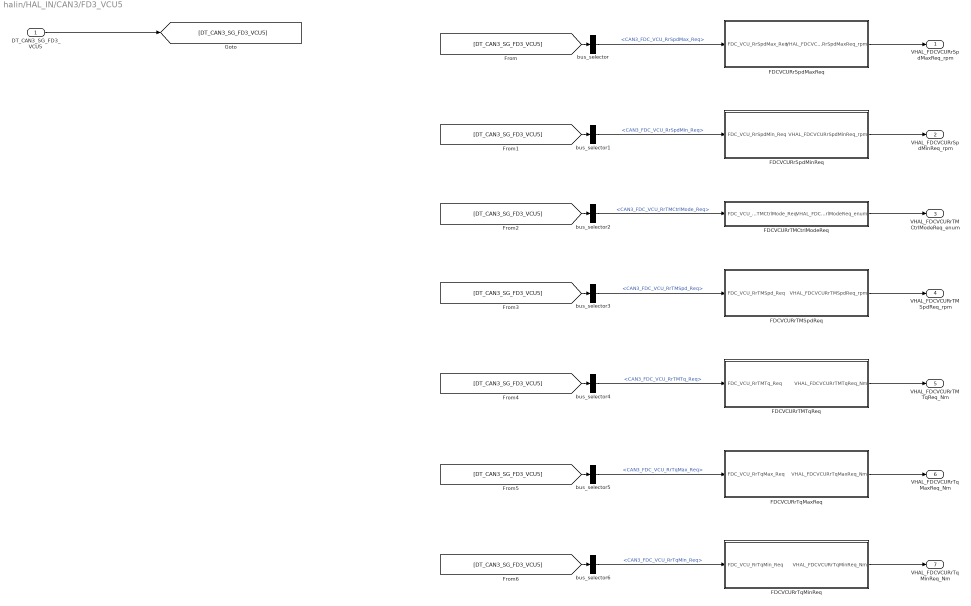
== system halin/HAL_IN/CAN3/FD3_VCU5 ==
  DT_CAN3_SG_FD3_VCU5 : Inport
  FDCVCURrSpdMaxReq : Subsystem
  FDCVCURrSpdMinReq : Subsystem
  FDCVCURrTMCtrlModeReq : Subsystem
  FDCVCURrTMSpdReq : Subsystem
  FDCVCURrTMTqReq : Subsystem
  FDCVCURrTqMaxReq : Subsystem
  FDCVCURrTqMinReq : Subsystem
  bus_selector : BusSelector  OutputSignals=CAN3_FDC_VCU_RrSpdMax_Req
  bus_selector1 : BusSelector  OutputSignals=CAN3_FDC_VCU_RrSpdMin_Req
  bus_selector2 : BusSelector  OutputSignals=CAN3_FDC_VCU_RrTMCtrlMode_Req
  bus_selector3 : BusSelector  OutputSignals=CAN3_FDC_VCU_RrTMSpd_Req
  bus_selector4 : BusSelector  OutputSignals=CAN3_FDC_VCU_RrTMTq_Req
  bus_selector5 : BusSelector  OutputSignals=CAN3_FDC_VCU_RrTqMax_Req
  bus_selector6 : BusSelector  OutputSignals=CAN3_FDC_VCU_RrTqMin_Req
  VHAL_FDCVCURrSpdMaxReq_rpm : Outport
  VHAL_FDCVCURrSpdMinReq_rpm : Outport  Port=2
  VHAL_FDCVCURrTMCtrlModeReq_enum : Outport  Port=3
  VHAL_FDCVCURrTMSpdReq_rpm : Outport  Port=4
  VHAL_FDCVCURrTMTqReq_Nm : Outport  Port=5
  VHAL_FDCVCURrTqMaxReq_Nm : Outport  Port=6
  VHAL_FDCVCURrTqMinReq_Nm : Outport  Port=7
  wires:
  DT_CAN3_SG_FD3_VCU5/1 -> [DT_CAN3_SG_FD3_VCU5]
  [DT_CAN3_SG_FD3_VCU5] -> bus_selector/1
  bus_selector/1 -> FDCVCURrSpdMaxReq/1(FDC_VCU_RrSpdMax_Req)  "<CAN3_FDC_VCU_RrSpdMax_Req>"
  FDCVCURrSpdMaxReq/1(VHAL_FDCVCURrSpdMaxReq_rpm) -> VHAL_FDCVCURrSpdMaxReq_rpm/1
  [DT_CAN3_SG_FD3_VCU5] -> bus_selector1/1
  bus_selector1/1 -> FDCVCURrSpdMinReq/1(FDC_VCU_RrSpdMin_Req)  "<CAN3_FDC_VCU_RrSpdMin_Req>"
  FDCVCURrSpdMinReq/1(VHAL_FDCVCURrSpdMinReq_rpm) -> VHAL_FDCVCURrSpdMinReq_rpm/1
  [DT_CAN3_SG_FD3_VCU5] -> bus_selector2/1
  bus_selector2/1 -> FDCVCURrTMCtrlModeReq/1(FDC_VCU_RrTMCtrlMode_Req)  "<CAN3_FDC_VCU_RrTMCtrlMode_Req>"
  FDCVCURrTMCtrlModeReq/1(VHAL_FDCVCURrTMCtrlModeReq_enum) -> VHAL_FDCVCURrTMCtrlModeReq_enum/1
  [DT_CAN3_SG_FD3_VCU5] -> bus_selector3/1
  bus_selector3/1 -> FDCVCURrTMSpdReq/1(FDC_VCU_RrTMSpd_Req)  "<CAN3_FDC_VCU_RrTMSpd_Req>"
  FDCVCURrTMSpdReq/1(VHAL_FDCVCURrTMSpdReq_rpm) -> VHAL_FDCVCURrTMSpdReq_rpm/1
  [DT_CAN3_SG_FD3_VCU5] -> bus_selector4/1
  bus_selector4/1 -> FDCVCURrTMTqReq/1(FDC_VCU_RrTMTq_Req)  "<CAN3_FDC_VCU_RrTMTq_Req>"
  FDCVCURrTMTqReq/1(VHAL_FDCVCURrTMTqReq_Nm) -> VHAL_FDCVCURrTMTqReq_Nm/1
  [DT_CAN3_SG_FD3_VCU5] -> bus_selector5/1
  bus_selector5/1 -> FDCVCURrTqMaxReq/1(FDC_VCU_RrTqMax_Req)  "<CAN3_FDC_VCU_RrTqMax_Req>"
  FDCVCURrTqMaxReq/1(VHAL_FDCVCURrTqMaxReq_Nm) -> VHAL_FDCVCURrTqMaxReq_Nm/1
  [DT_CAN3_SG_FD3_VCU5] -> bus_selector6/1
  bus_selector6/1 -> FDCVCURrTqMinReq/1(FDC_VCU_RrTqMin_Req)  "<CAN3_FDC_VCU_RrTqMin_Req>"
  FDCVCURrTqMinReq/1(VHAL_FDCVCURrTqMinReq_Nm) -> VHAL_FDCVCURrTqMinReq_Nm/1

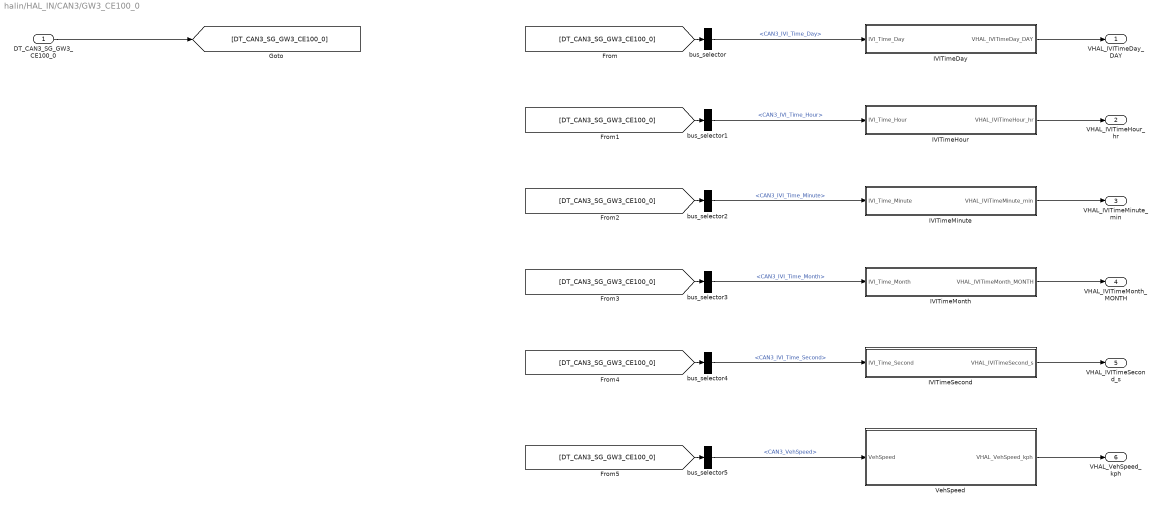
== system halin/HAL_IN/CAN3/GW3_CE100_0 ==
  DT_CAN3_SG_GW3_CE100_0 : Inport
  IVITimeDay : Subsystem
  IVITimeHour : Subsystem
  IVITimeMinute : Subsystem
  IVITimeMonth : Subsystem
  IVITimeSecond : Subsystem
  VehSpeed : Subsystem
  bus_selector : BusSelector  OutputSignals=CAN3_IVI_Time_Day
  bus_selector1 : BusSelector  OutputSignals=CAN3_IVI_Time_Hour
  bus_selector2 : BusSelector  OutputSignals=CAN3_IVI_Time_Minute
  bus_selector3 : BusSelector  OutputSignals=CAN3_IVI_Time_Month
  bus_selector4 : BusSelector  OutputSignals=CAN3_IVI_Time_Second
  bus_selector5 : BusSelector  OutputSignals=CAN3_VehSpeed
  VHAL_IVITimeDay_DAY : Outport
  VHAL_IVITimeHour_hr : Outport  Port=2
  VHAL_IVITimeMinute_min : Outport  Port=3
  VHAL_IVITimeMonth_MONTH : Outport  Port=4
  VHAL_IVITimeSecond_s : Outport  Port=5
  VHAL_VehSpeed_kph : Outport  Port=6
  wires:
  DT_CAN3_SG_GW3_CE100_0/1 -> [DT_CAN3_SG_GW3_CE100_0]
  [DT_CAN3_SG_GW3_CE100_0] -> bus_selector/1
  bus_selector/1 -> IVITimeDay/1(IVI_Time_Day)  "<CAN3_IVI_Time_Day>"
  IVITimeDay/1(VHAL_IVITimeDay_DAY) -> VHAL_IVITimeDay_DAY/1
  [DT_CAN3_SG_GW3_CE100_0] -> bus_selector1/1
  bus_selector1/1 -> IVITimeHour/1(IVI_Time_Hour)  "<CAN3_IVI_Time_Hour>"
  IVITimeHour/1(VHAL_IVITimeHour_hr) -> VHAL_IVITimeHour_hr/1
  [DT_CAN3_SG_GW3_CE100_0] -> bus_selector2/1
  bus_selector2/1 -> IVITimeMinute/1(IVI_Time_Minute)  "<CAN3_IVI_Time_Minute>"
  IVITimeMinute/1(VHAL_IVITimeMinute_min) -> VHAL_IVITimeMinute_min/1
  [DT_CAN3_SG_GW3_CE100_0] -> bus_selector3/1
  bus_selector3/1 -> IVITimeMonth/1(IVI_Time_Month)  "<CAN3_IVI_Time_Month>"
  IVITimeMonth/1(VHAL_IVITimeMonth_MONTH) -> VHAL_IVITimeMonth_MONTH/1
  [DT_CAN3_SG_GW3_CE100_0] -> bus_selector4/1
  bus_selector4/1 -> IVITimeSecond/1(IVI_Time_Second)  "<CAN3_IVI_Time_Second>"
  IVITimeSecond/1(VHAL_IVITimeSecond_s) -> VHAL_IVITimeSecond_s/1
  [DT_CAN3_SG_GW3_CE100_0] -> bus_selector5/1
  bus_selector5/1 -> VehSpeed/1(VehSpeed)  "<CAN3_VehSpeed>"
  VehSpeed/1(VHAL_VehSpeed_kph) -> VHAL_VehSpeed_kph/1

== system halin/HAL_IN/CAN_MCU_R1/CheckTimeoutSubsystem ==
  EOP_FVT_R_Local1_Status : Inport
  Equal : RelationalOperator  Operator===  OutDataTypeStr=boolean  RndMeth=Simplest  InputSameDT=off
  constant : Constant  Value=TimeoutOccurred
  VHAL_CANMsgInvalidEOPFVTRLocal1_flg : Outport
  wires:
  EOP_FVT_R_Local1_Status/1 -> Equal/1
  constant/1 -> Equal/2
  Equal/1 -> VHAL_CANMsgInvalidEOPFVTRLocal1_flg/1  "VHAL_CANMsgInvalidEOPFVTRLocal1_flg"

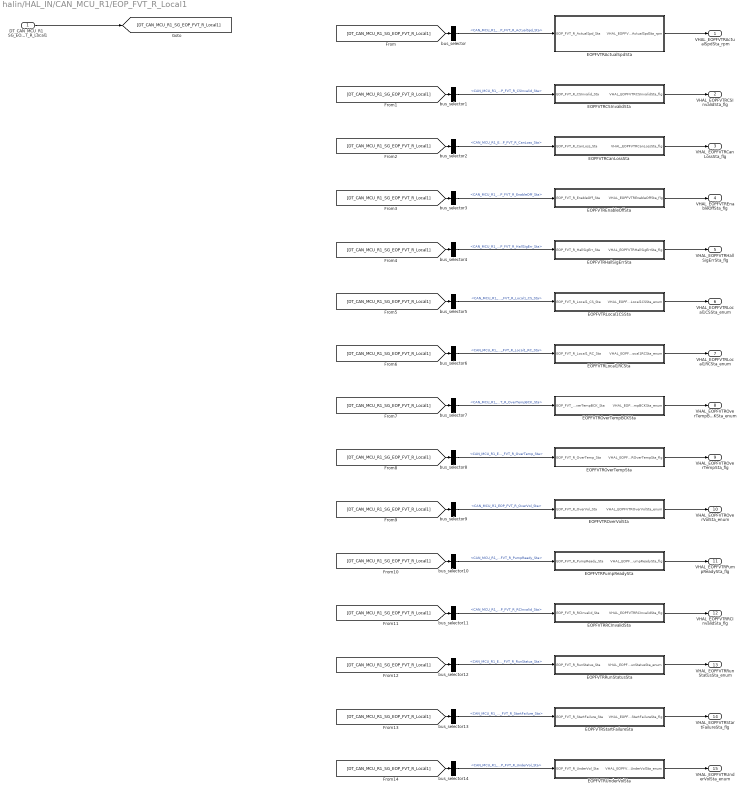
== system halin/HAL_IN/CAN_MCU_R1/EOP_FVT_R_Local1 ==
  DT_CAN_MCU_R1_SG_EOP_FVT_R_Local1 : Inport
  EOPFVTRActualSpdSta : Subsystem
  EOPFVTRCSInvalidSta : Subsystem
  EOPFVTRCanLossSta : Subsystem
  EOPFVTREnableOffSta : Subsystem
  EOPFVTRHallSigErrSta : Subsystem
  EOPFVTRLocal1CSSta : Subsystem
  EOPFVTRLocal1RCSta : Subsystem
  EOPFVTROverTempBCKSta : Subsystem
  EOPFVTROverTempSta : Subsystem
  EOPFVTROverVolSta : Subsystem
  EOPFVTRPumpReadySta : Subsystem
  EOPFVTRRCInvalidSta : Subsystem
  EOPFVTRRunStatusSta : Subsystem
  EOPFVTRStartFailureSta : Subsystem
  EOPFVTRUnderVolSta : Subsystem
  bus_selector : BusSelector  OutputSignals=CAN_MCU_R1_EOP_FVT_R_ActualSpd_Sta
  bus_selector1 : BusSelector  OutputSignals=CAN_MCU_R1_EOP_FVT_R_CSInvalid_Sta
  bus_selector10 : BusSelector  OutputSignals=CAN_MCU_R1_EOP_FVT_R_PumpReady_Sta
  bus_selector11 : BusSelector  OutputSignals=CAN_MCU_R1_EOP_FVT_R_RCInvalid_Sta
  bus_selector12 : BusSelector  OutputSignals=CAN_MCU_R1_EOP_FVT_R_RunStatus_Sta
  bus_selector13 : BusSelector  OutputSignals=CAN_MCU_R1_EOP_FVT_R_StartFailure_Sta
  bus_selector14 : BusSelector  OutputSignals=CAN_MCU_R1_EOP_FVT_R_UnderVol_Sta
  bus_selector2 : BusSelector  OutputSignals=CAN_MCU_R1_EOP_FVT_R_CanLoss_Sta
  bus_selector3 : BusSelector  OutputSignals=CAN_MCU_R1_EOP_FVT_R_EnableOff_Sta
  bus_selector4 : BusSelector  OutputSignals=CAN_MCU_R1_EOP_FVT_R_HallSigErr_Sta
  bus_selector5 : BusSelector  OutputSignals=CAN_MCU_R1_EOP_FVT_R_Local1_CS_Sta
  bus_selector6 : BusSelector  OutputSignals=CAN_MCU_R1_EOP_FVT_R_Local1_RC_Sta
  bus_selector7 : BusSelector  OutputSignals=CAN_MCU_R1_EOP_FVT_R_OverTempBCK_Sta
  bus_selector8 : BusSelector  OutputSignals=CAN_MCU_R1_EOP_FVT_R_OverTemp_Sta
  bus_selector9 : BusSelector  OutputSignals=CAN_MCU_R1_EOP_FVT_R_OverVol_Sta
  VHAL_EOPFVTRActualSpdSta_rpm : Outport
  VHAL_EOPFVTRCSInvalidSta_flg : Outport  Port=2
  VHAL_EOPFVTRCanLossSta_flg : Outport  Port=3
  VHAL_EOPFVTREnableOffSta_flg : Outport  Port=4
  VHAL_EOPFVTRHallSigErrSta_flg : Outport  Port=5
  VHAL_EOPFVTRLocal1CSSta_enum : Outport  Port=6
  VHAL_EOPFVTRLocal1RCSta_enum : Outport  Port=7
  VHAL_EOPFVTROverTempBCKSta_enum : Outport  Port=8
  VHAL_EOPFVTROverTempSta_flg : Outport  Port=9
  VHAL_EOPFVTROverVolSta_enum : Outport  Port=10
  VHAL_EOPFVTRPumpReadySta_flg : Outport  Port=11
  VHAL_EOPFVTRRCInvalidSta_flg : Outport  Port=12
  VHAL_EOPFVTRRunStatusSta_enum : Outport  Port=13
  VHAL_EOPFVTRStartFailureSta_flg : Outport  Port=14
  VHAL_EOPFVTRUnderVolSta_enum : Outport  Port=15
  wires:
  DT_CAN_MCU_R1_SG_EOP_FVT_R_Local1/1 -> [DT_CAN_MCU_R1_SG_EOP_FVT_R_Local1]
  [DT_CAN_MCU_R1_SG_EOP_FVT_R_Local1] -> bus_selector/1
  bus_selector/1 -> EOPFVTRActualSpdSta/1(EOP_FVT_R_ActualSpd_Sta)  "<CAN_MCU_R1_EOP_FVT_R_ActualSpd_Sta>"
  EOPFVTRActualSpdSta/1(VHAL_EOPFVTRActualSpdSta_rpm) -> VHAL_EOPFVTRActualSpdSta_rpm/1
  [DT_CAN_MCU_R1_SG_EOP_FVT_R_Local1] -> bus_selector1/1
  bus_selector1/1 -> EOPFVTRCSInvalidSta/1(EOP_FVT_R_CSInvalid_Sta)  "<CAN_MCU_R1_EOP_FVT_R_CSInvalid_Sta>"
  EOPFVTRCSInvalidSta/1(VHAL_EOPFVTRCSInvalidSta_flg) -> VHAL_EOPFVTRCSInvalidSta_flg/1
  [DT_CAN_MCU_R1_SG_EOP_FVT_R_Local1] -> bus_selector2/1
  bus_selector2/1 -> EOPFVTRCanLossSta/1(EOP_FVT_R_CanLoss_Sta)  "<CAN_MCU_R1_EOP_FVT_R_CanLoss_Sta>"
  EOPFVTRCanLossSta/1(VHAL_EOPFVTRCanLossSta_flg) -> VHAL_EOPFVTRCanLossSta_flg/1
  [DT_CAN_MCU_R1_SG_EOP_FVT_R_Local1] -> bus_selector3/1
  bus_selector3/1 -> EOPFVTREnableOffSta/1(EOP_FVT_R_EnableOff_Sta)  "<CAN_MCU_R1_EOP_FVT_R_EnableOff_Sta>"
  EOPFVTREnableOffSta/1(VHAL_EOPFVTREnableOffSta_flg) -> VHAL_EOPFVTREnableOffSta_flg/1
  [DT_CAN_MCU_R1_SG_EOP_FVT_R_Local1] -> bus_selector4/1
  bus_selector4/1 -> EOPFVTRHallSigErrSta/1(EOP_FVT_R_HallSigErr_Sta)  "<CAN_MCU_R1_EOP_FVT_R_HallSigErr_Sta>"
  EOPFVTRHallSigErrSta/1(VHAL_EOPFVTRHallSigErrSta_flg) -> VHAL_EOPFVTRHallSigErrSta_flg/1
  [DT_CAN_MCU_R1_SG_EOP_FVT_R_Local1] -> bus_selector5/1
  bus_selector5/1 -> EOPFVTRLocal1CSSta/1(EOP_FVT_R_Local1_CS_Sta)  "<CAN_MCU_R1_EOP_FVT_R_Local1_CS_Sta>"
  EOPFVTRLocal1CSSta/1(VHAL_EOPFVTRLocal1CSSta_enum) -> VHAL_EOPFVTRLocal1CSSta_enum/1
  [DT_CAN_MCU_R1_SG_EOP_FVT_R_Local1] -> bus_selector6/1
  bus_selector6/1 -> EOPFVTRLocal1RCSta/1(EOP_FVT_R_Local1_RC_Sta)  "<CAN_MCU_R1_EOP_FVT_R_Local1_RC_Sta>"
  EOPFVTRLocal1RCSta/1(VHAL_EOPFVTRLocal1RCSta_enum) -> VHAL_EOPFVTRLocal1RCSta_enum/1
  [DT_CAN_MCU_R1_SG_EOP_FVT_R_Local1] -> bus_selector7/1
  bus_selector7/1 -> EOPFVTROverTempBCKSta/1(EOP_FVT_R_OverTempBCK_Sta)  "<CAN_MCU_R1_EOP_FVT_R_OverTempBCK_Sta>"
  EOPFVTROverTempBCKSta/1(VHAL_EOPFVTROverTempBCKSta_enum) -> VHAL_EOPFVTROverTempBCKSta_enum/1
  [DT_CAN_MCU_R1_SG_EOP_FVT_R_Local1] -> bus_selector8/1
  bus_selector8/1 -> EOPFVTROverTempSta/1(EOP_FVT_R_OverTemp_Sta)  "<CAN_MCU_R1_EOP_FVT_R_OverTemp_Sta>"
  EOPFVTROverTempSta/1(VHAL_EOPFVTROverTempSta_flg) -> VHAL_EOPFVTROverTempSta_flg/1
  [DT_CAN_MCU_R1_SG_EOP_FVT_R_Local1] -> bus_selector9/1
  bus_selector9/1 -> EOPFVTROverVolSta/1(EOP_FVT_R_OverVol_Sta)  "<CAN_MCU_R1_EOP_FVT_R_OverVol_Sta>"
  EOPFVTROverVolSta/1(VHAL_EOPFVTROverVolSta_enum) -> VHAL_EOPFVTROverVolSta_enum/1
  [DT_CAN_MCU_R1_SG_EOP_FVT_R_Local1] -> bus_selector10/1
  bus_selector10/1 -> EOPFVTRPumpReadySta/1(EOP_FVT_R_PumpReady_Sta)  "<CAN_MCU_R1_EOP_FVT_R_PumpReady_Sta>"
  EOPFVTRPumpReadySta/1(VHAL_EOPFVTRPumpReadySta_flg) -> VHAL_EOPFVTRPumpReadySta_flg/1
  [DT_CAN_MCU_R1_SG_EOP_FVT_R_Local1] -> bus_selector11/1
  bus_selector11/1 -> EOPFVTRRCInvalidSta/1(EOP_FVT_R_RCInvalid_Sta)  "<CAN_MCU_R1_EOP_FVT_R_RCInvalid_Sta>"
  EOPFVTRRCInvalidSta/1(VHAL_EOPFVTRRCInvalidSta_flg) -> VHAL_EOPFVTRRCInvalidSta_flg/1
  [DT_CAN_MCU_R1_SG_EOP_FVT_R_Local1] -> bus_selector12/1
  bus_selector12/1 -> EOPFVTRRunStatusSta/1(EOP_FVT_R_RunStatus_Sta)  "<CAN_MCU_R1_EOP_FVT_R_RunStatus_Sta>"
  EOPFVTRRunStatusSta/1(VHAL_EOPFVTRRunStatusSta_enum) -> VHAL_EOPFVTRRunStatusSta_enum/1
  [DT_CAN_MCU_R1_SG_EOP_FVT_R_Local1] -> bus_selector13/1
  bus_selector13/1 -> EOPFVTRStartFailureSta/1(EOP_FVT_R_StartFailure_Sta)  "<CAN_MCU_R1_EOP_FVT_R_StartFailure_Sta>"
  EOPFVTRStartFailureSta/1(VHAL_EOPFVTRStartFailureSta_flg) -> VHAL_EOPFVTRStartFailureSta_flg/1
  [DT_CAN_MCU_R1_SG_EOP_FVT_R_Local1] -> bus_selector14/1
  bus_selector14/1 -> EOPFVTRUnderVolSta/1(EOP_FVT_R_UnderVol_Sta)  "<CAN_MCU_R1_EOP_FVT_R_UnderVol_Sta>"
  EOPFVTRUnderVolSta/1(VHAL_EOPFVTRUnderVolSta_enum) -> VHAL_EOPFVTRUnderVolSta_enum/1

== system halin/HAL_IN/CAN3/BMS1/HVBattVolt ==
  HVBattVolt : Inport
  UnitConverter : DataTypeConversion  OutDataTypeStr=uint16  SaturateOnIntegerOverflow=off  RndMeth=Floor
  convert_in : FVT_lib/hal/convert_in  gain=0.1  offset=0
  VHAL_HVBattVolt_V : Outport
  wires:
  convert_in/1 -> VHAL_HVBattVolt_V/1
  UnitConverter/1 -> convert_in/1
  HVBattVolt/1 -> UnitConverter/1

== system halin/HAL_IN/CAN3/BMS6/HVBContactorSta ==
  HVBContactorSta : Inport
  UnitConverter : DataTypeConversion  OutDataTypeStr=uint8  SaturateOnIntegerOverflow=off  RndMeth=Floor
  VHAL_HVBContactorSta_flg : Outport
  wires:
  UnitConverter/1 -> VHAL_HVBContactorSta_flg/1
  HVBContactorSta/1 -> UnitConverter/1

== system halin/HAL_IN/CAN3/FD3_C100_0/BatteryMode ==
  BatteryMode : Inport
  UnitConverter : DataTypeConversion  OutDataTypeStr=uint8  SaturateOnIntegerOverflow=off  RndMeth=Floor
  VHAL_BatteryMode_enum : Outport
  wires:
  UnitConverter/1 -> VHAL_BatteryMode_enum/1
  BatteryMode/1 -> UnitConverter/1

== system halin/HAL_IN/CAN3/FD3_C100_0/RrCoolantflow ==
  Rr_Coolantflow : Inport
  UnitConverter : DataTypeConversion  OutDataTypeStr=uint8  SaturateOnIntegerOverflow=off  RndMeth=Floor
  convert_in : FVT_lib/hal/convert_in  gain=0.25  offset=0
  VHAL_RrCoolantflow_Lpmin : Outport
  wires:
  convert_in/1 -> VHAL_RrCoolantflow_Lpmin/1
  UnitConverter/1 -> convert_in/1
  Rr_Coolantflow/1 -> UnitConverter/1

== system halin/HAL_IN/CAN3/FD3_C100_0/RrCoolanttemp ==
  Rr_Coolanttemp : Inport
  UnitConverter : DataTypeConversion  OutDataTypeStr=uint16  SaturateOnIntegerOverflow=off  RndMeth=Floor
  convert_in : FVT_lib/hal/convert_in  gain=1  offset=-40
  VHAL_RrCoolanttemp_C : Outport
  wires:
  convert_in/1 -> VHAL_RrCoolanttemp_C/1
  UnitConverter/1 -> convert_in/1
  Rr_Coolanttemp/1 -> UnitConverter/1

== system halin/HAL_IN/CAN3/FD3_VCU1/ActiveDischReq ==
  ActiveDischReq : Inport
  UnitConverter : DataTypeConversion  OutDataTypeStr=uint8  SaturateOnIntegerOverflow=off  RndMeth=Floor
  VHAL_ActiveDischReq_flg : Outport
  wires:
  UnitConverter/1 -> VHAL_ActiveDischReq_flg/1
  ActiveDischReq/1 -> UnitConverter/1

== system halin/HAL_IN/CAN3/FD3_VCU1/CSVCU1 ==
  CS_VCU1 : Inport
  UnitConverter : DataTypeConversion  OutDataTypeStr=uint8  SaturateOnIntegerOverflow=off  RndMeth=Floor
  VHAL_CSVCU1_enum : Outport
  wires:
  UnitConverter/1 -> VHAL_CSVCU1_enum/1
  CS_VCU1/1 -> UnitConverter/1

== system halin/HAL_IN/CAN3/FD3_VCU1/PwrSta ==
  PwrSta : Inport
  UnitConverter : DataTypeConversion  OutDataTypeStr=uint8  SaturateOnIntegerOverflow=off  RndMeth=Floor
  VHAL_PwrSta_enum : Outport
  wires:
  UnitConverter/1 -> VHAL_PwrSta_enum/1
  PwrSta/1 -> UnitConverter/1

== system halin/HAL_IN/CAN3/FD3_VCU1/RCVCU1 ==
  RC_VCU1 : Inport
  UnitConverter : DataTypeConversion  OutDataTypeStr=uint8  SaturateOnIntegerOverflow=off  RndMeth=Floor
  VHAL_RCVCU1_enum : Outport
  wires:
  UnitConverter/1 -> VHAL_RCVCU1_enum/1
  RC_VCU1/1 -> UnitConverter/1

== system halin/HAL_IN/CAN3/FD3_VCU1/ShiftGearPosn ==
  ShiftGearPosn : Inport
  UnitConverter : DataTypeConversion  OutDataTypeStr=uint8  SaturateOnIntegerOverflow=off  RndMeth=Floor
  VHAL_ShiftGearPosn_enum : Outport
  wires:
  UnitConverter/1 -> VHAL_ShiftGearPosn_enum/1
  ShiftGearPosn/1 -> UnitConverter/1

== system halin/HAL_IN/CAN3/FD3_VCU2/CSVCU2CAN1 ==
  CS_VCU2_CAN1 : Inport
  UnitConverter : DataTypeConversion  OutDataTypeStr=uint8  SaturateOnIntegerOverflow=off  RndMeth=Floor
  VHAL_CSVCU2CAN1_enum : Outport
  wires:
  UnitConverter/1 -> VHAL_CSVCU2CAN1_enum/1
  CS_VCU2_CAN1/1 -> UnitConverter/1

== system halin/HAL_IN/CAN3/FD3_VCU2/RCVCU2CAN1 ==
  RC_VCU2_CAN1 : Inport
  UnitConverter : DataTypeConversion  OutDataTypeStr=uint8  SaturateOnIntegerOverflow=off  RndMeth=Floor
  VHAL_RCVCU2CAN1_enum : Outport
  wires:
  UnitConverter/1 -> VHAL_RCVCU2CAN1_enum/1
  RC_VCU2_CAN1/1 -> UnitConverter/1

== system halin/HAL_IN/CAN3/FD3_VCU2/RrActvDmpDisabReq ==
  Rr_ActvDmpDisabReq : Inport
  UnitConverter : DataTypeConversion  OutDataTypeStr=uint8  SaturateOnIntegerOverflow=off  RndMeth=Floor
  VHAL_RrActvDmpDisabReq_flg : Outport
  wires:
  UnitConverter/1 -> VHAL_RrActvDmpDisabReq_flg/1
  Rr_ActvDmpDisabReq/1 -> UnitConverter/1

== system halin/HAL_IN/CAN3/FD3_VCU2/RrMCUEnaReq ==
  Rr_MCUEnaReq : Inport
  UnitConverter : DataTypeConversion  OutDataTypeStr=uint8  SaturateOnIntegerOverflow=off  RndMeth=Floor
  VHAL_RrMCUEnaReq_flg : Outport
  wires:
  UnitConverter/1 -> VHAL_RrMCUEnaReq_flg/1
  Rr_MCUEnaReq/1 -> UnitConverter/1

== system halin/HAL_IN/CAN3/FD3_VCU5/FDCVCURrSpdMaxReq ==
  FDC_VCU_RrSpdMax_Req : Inport
  UnitConverter : DataTypeConversion  OutDataTypeStr=uint16  SaturateOnIntegerOverflow=off  RndMeth=Floor
  VHAL_FDCVCURrSpdMaxReq_rpm : Outport
  wires:
  UnitConverter/1 -> VHAL_FDCVCURrSpdMaxReq_rpm/1
  FDC_VCU_RrSpdMax_Req/1 -> UnitConverter/1

== system halin/HAL_IN/CAN3/FD3_VCU5/FDCVCURrSpdMinReq ==
  FDC_VCU_RrSpdMin_Req : Inport
  UnitConverter : DataTypeConversion  OutDataTypeStr=uint16  SaturateOnIntegerOverflow=off  RndMeth=Floor
  convert_in : FVT_lib/hal/convert_in  gain=1  offset=-22000
  VHAL_FDCVCURrSpdMinReq_rpm : Outport
  wires:
  convert_in/1 -> VHAL_FDCVCURrSpdMinReq_rpm/1
  UnitConverter/1 -> convert_in/1
  FDC_VCU_RrSpdMin_Req/1 -> UnitConverter/1

== system halin/HAL_IN/CAN3/FD3_VCU5/FDCVCURrTMCtrlModeReq ==
  FDC_VCU_RrTMCtrlMode_Req : Inport
  UnitConverter : DataTypeConversion  OutDataTypeStr=uint8  SaturateOnIntegerOverflow=off  RndMeth=Floor
  VHAL_FDCVCURrTMCtrlModeReq_enum : Outport
  wires:
  UnitConverter/1 -> VHAL_FDCVCURrTMCtrlModeReq_enum/1
  FDC_VCU_RrTMCtrlMode_Req/1 -> UnitConverter/1

== system halin/HAL_IN/CAN3/FD3_VCU5/FDCVCURrTMSpdReq ==
  FDC_VCU_RrTMSpd_Req : Inport
  UnitConverter : DataTypeConversion  OutDataTypeStr=uint16  SaturateOnIntegerOverflow=off  RndMeth=Floor
  convert_in : FVT_lib/hal/convert_in  gain=1  offset=-22000
  VHAL_FDCVCURrTMSpdReq_rpm : Outport
  wires:
  convert_in/1 -> VHAL_FDCVCURrTMSpdReq_rpm/1
  UnitConverter/1 -> convert_in/1
  FDC_VCU_RrTMSpd_Req/1 -> UnitConverter/1

== system halin/HAL_IN/CAN3/FD3_VCU5/FDCVCURrTMTqReq ==
  FDC_VCU_RrTMTq_Req : Inport
  UnitConverter : DataTypeConversion  OutDataTypeStr=uint16  SaturateOnIntegerOverflow=off  RndMeth=Floor
  convert_in : FVT_lib/hal/convert_in  gain=0.1  offset=-1000
  VHAL_FDCVCURrTMTqReq_Nm : Outport
  wires:
  convert_in/1 -> VHAL_FDCVCURrTMTqReq_Nm/1
  UnitConverter/1 -> convert_in/1
  FDC_VCU_RrTMTq_Req/1 -> UnitConverter/1

== system halin/HAL_IN/CAN3/FD3_VCU5/FDCVCURrTqMaxReq ==
  FDC_VCU_RrTqMax_Req : Inport
  UnitConverter : DataTypeConversion  OutDataTypeStr=uint16  SaturateOnIntegerOverflow=off  RndMeth=Floor
  VHAL_FDCVCURrTqMaxReq_Nm : Outport
  wires:
  UnitConverter/1 -> VHAL_FDCVCURrTqMaxReq_Nm/1
  FDC_VCU_RrTqMax_Req/1 -> UnitConverter/1

== system halin/HAL_IN/CAN3/FD3_VCU5/FDCVCURrTqMinReq ==
  FDC_VCU_RrTqMin_Req : Inport
  UnitConverter : DataTypeConversion  OutDataTypeStr=uint16  SaturateOnIntegerOverflow=off  RndMeth=Floor
  convert_in : FVT_lib/hal/convert_in  gain=1  offset=-1022
  VHAL_FDCVCURrTqMinReq_Nm : Outport
  wires:
  convert_in/1 -> VHAL_FDCVCURrTqMinReq_Nm/1
  UnitConverter/1 -> convert_in/1
  FDC_VCU_RrTqMin_Req/1 -> UnitConverter/1

== system halin/HAL_IN/CAN3/GW3_CE100_0/IVITimeDay ==
  IVI_Time_Day : Inport
  UnitConverter : DataTypeConversion  OutDataTypeStr=uint8  SaturateOnIntegerOverflow=off  RndMeth=Floor
  VHAL_IVITimeDay_DAY : Outport
  wires:
  UnitConverter/1 -> VHAL_IVITimeDay_DAY/1
  IVI_Time_Day/1 -> UnitConverter/1

== system halin/HAL_IN/CAN3/GW3_CE100_0/IVITimeHour ==
  IVI_Time_Hour : Inport
  UnitConverter : DataTypeConversion  OutDataTypeStr=uint8  SaturateOnIntegerOverflow=off  RndMeth=Floor
  VHAL_IVITimeHour_hr : Outport
  wires:
  UnitConverter/1 -> VHAL_IVITimeHour_hr/1
  IVI_Time_Hour/1 -> UnitConverter/1

== system halin/HAL_IN/CAN3/GW3_CE100_0/IVITimeMinute ==
  IVI_Time_Minute : Inport
  UnitConverter : DataTypeConversion  OutDataTypeStr=uint8  SaturateOnIntegerOverflow=off  RndMeth=Floor
  VHAL_IVITimeMinute_min : Outport
  wires:
  UnitConverter/1 -> VHAL_IVITimeMinute_min/1
  IVI_Time_Minute/1 -> UnitConverter/1

== system halin/HAL_IN/CAN3/GW3_CE100_0/IVITimeMonth ==
  IVI_Time_Month : Inport
  UnitConverter : DataTypeConversion  OutDataTypeStr=uint8  SaturateOnIntegerOverflow=off  RndMeth=Floor
  VHAL_IVITimeMonth_MONTH : Outport
  wires:
  UnitConverter/1 -> VHAL_IVITimeMonth_MONTH/1
  IVI_Time_Month/1 -> UnitConverter/1

== system halin/HAL_IN/CAN3/GW3_CE100_0/IVITimeSecond ==
  IVI_Time_Second : Inport
  UnitConverter : DataTypeConversion  OutDataTypeStr=uint8  SaturateOnIntegerOverflow=off  RndMeth=Floor
  VHAL_IVITimeSecond_s : Outport
  wires:
  UnitConverter/1 -> VHAL_IVITimeSecond_s/1
  IVI_Time_Second/1 -> UnitConverter/1

== system halin/HAL_IN/CAN3/GW3_CE100_0/VehSpeed ==
  VehSpeed : Inport
  UnitConverter : DataTypeConversion  OutDataTypeStr=uint16  SaturateOnIntegerOverflow=off  RndMeth=Floor
  convert_in : FVT_lib/hal/convert_in  gain=0.125  offset=0
  VHAL_VehSpeed_kph : Outport
  wires:
  convert_in/1 -> VHAL_VehSpeed_kph/1
  UnitConverter/1 -> convert_in/1
  VehSpeed/1 -> UnitConverter/1
